simulink library "Cassie_CommandBlock_Library_6"  (R2017b)
settings: Solver=VariableStepAuto  StartTime=0.0  StopTime=10.0  RelTol=1e-3
undefined symbols (not defined in the file): dq, isSim, q, sample_time
libraries: slrtlib x119, Cassie_CommandBlock_Library_5 x1
(part 2 of 3)

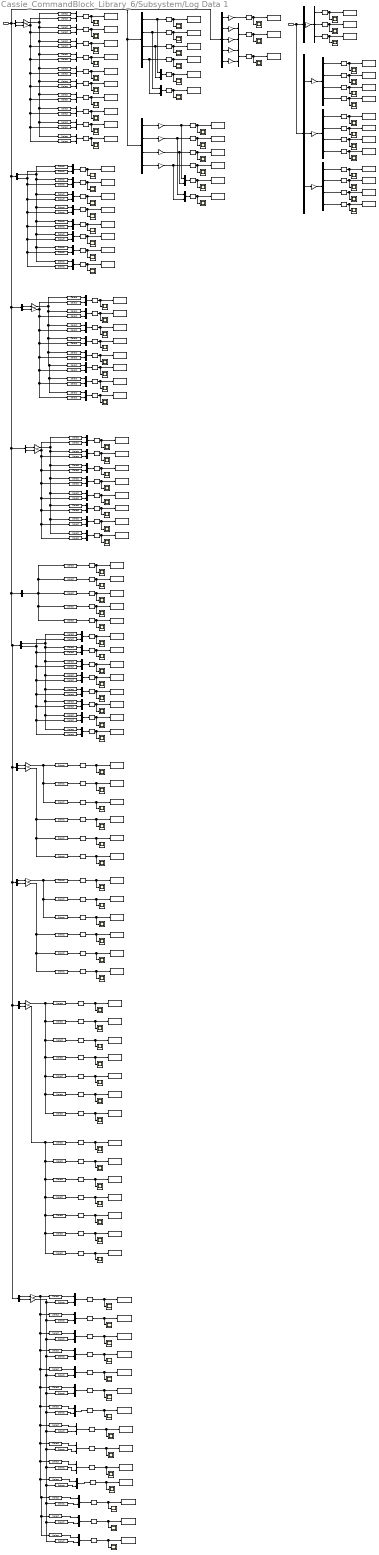
== system Cassie_CommandBlock_Library_6/Subsystem/Log Data 1 ==
  In1 : Inport
  In2 : Inport  Port=2  OutDataTypeStr=Bus: StateEstimator_DataBus
  Bus Selector : BusSelector  OutputSignals=qm0,qmd
  Bus Selector1 : BusSelector  OutputSignals=hr,hr_recover
  Bus Selector10 : BusSelector  OutputSignals=rp_LToe,rp_RToe,rp_LToe_fil,rp_RToe_fil
  Bus Selector11 : BusSelector  OutputSignals=s,qsL_1,qsR_1,qsL_2,qsR_2
  Bus Selector12 : BusSelector  OutputSignals=dq,dq_ss
  Bus Selector13 : BusSelector  OutputSignals=a_world
  Bus Selector14 : BusSelector  OutputSignals=ITx_kf,ITy_kf,ITz_kf
  Bus Selector2 : BusSelector  OutputSignals=hr,h0
  Bus Selector3 : BusSelector  OutputSignals=qd_control,q0_control
  Bus Selector4 : BusSelector  OutputSignals=dqd_control,dq0_control
  Bus Selector5 : BusSelector  OutputSignals=u
  Bus Selector6 : BusSelector  OutputSignals=q,dq
  Bus Selector7 : BusSelector  OutputSignals=q,dq
  Bus Selector8 : BusSelector  OutputSignals=q,dq
  Bus Selector9 : BusSelector  OutputSignals=Lx_stToe_stTD0_obs,Ly_stToe_stTD0_obs,Lx_stToe_stTD0_kf,Ly_stToe_stTD0_kf
  Demux : Demux  Outputs=3
  Demux1 : Demux
  Demux2 : Demux
  Demux3 : Demux
  Gain{,1..4,16..17,24..26} (10 alike) : Gain  Gain=1000
  Gain{5..8,10..15,18..23} (16 alike) : Gain  Gain=180/pi
  Gain9 : Gain  Gain=10
  Mux{,1..61} (62 alike) : Mux  Inputs=2
  Reshape{,1..116} (117 alike) : Reshape
  Scope{,1..116} (117 alike) : Scope
  "Scope " : slrtlib/Displays and Logging/Scope   scopeno=101  scopetype=Host  autostart=on  viewmode=Graphical redraw  formatstr='%15.6f'  grid=on  ylimits=[0,0]  nosamples=250  noprepostsamples=0  interleave=1  triggermode=FreeRun  triggersignal=1  trigsignalfromport=off  triggerlevel=0.0  triggerslope=Either  triggerscope=1  triggersample=0  filename=data.dat  mode=Lazy  writesize=512  autorestart=off  dynamicfilemode=off  maxwritefilesize=512*1024^2
  Scope 1 : slrtlib/Displays and Logging/Scope   scopeno=102  scopetype=Host  autostart=on  viewmode=Graphical redraw  formatstr='%15.6f'  grid=on  ylimits=[0,0]  nosamples=2500  noprepostsamples=0  interleave=1  triggermode=FreeRun  triggersignal=1  trigsignalfromport=off  triggerlevel=0.0  triggerslope=Either  triggerscope=1  triggersample=0  filename=data.dat  mode=Lazy  writesize=512  autorestart=off  dynamicfilemode=off  maxwritefilesize=512*1024^2
  Scope 10 : slrtlib/Displays and Logging/Scope   scopeno=111  scopetype=Host  autostart=on  viewmode=Graphical redraw  formatstr='%15.6f'  grid=on  ylimits=[0,0]  nosamples=2500  noprepostsamples=0  interleave=1  triggermode=FreeRun  triggersignal=1  trigsignalfromport=off  triggerlevel=0.0  triggerslope=Either  triggerscope=1  triggersample=0  filename=data.dat  mode=Lazy  writesize=512  autorestart=off  dynamicfilemode=off  maxwritefilesize=512*1024^2
  Scope 100 : slrtlib/Displays and Logging/Scope   scopeno=501  scopetype=Host  autostart=on  viewmode=Graphical redraw  formatstr='%15.6f'  grid=on  ylimits=[0,0]  nosamples=2500  noprepostsamples=0  interleave=1  triggermode=FreeRun  triggersignal=1  trigsignalfromport=off  triggerlevel=0.0  triggerslope=Either  triggerscope=1  triggersample=0  filename=data.dat  mode=Lazy  writesize=512  autorestart=off  dynamicfilemode=off  maxwritefilesize=512*1024^2
  Scope 101 : slrtlib/Displays and Logging/Scope   scopeno=502  scopetype=Host  autostart=on  viewmode=Graphical redraw  formatstr='%15.6f'  grid=on  ylimits=[0,0]  nosamples=2500  noprepostsamples=0  interleave=1  triggermode=FreeRun  triggersignal=1  trigsignalfromport=off  triggerlevel=0.0  triggerslope=Either  triggerscope=1  triggersample=0  filename=data.dat  mode=Lazy  writesize=512  autorestart=off  dynamicfilemode=off  maxwritefilesize=512*1024^2
  Scope 102 : slrtlib/Displays and Logging/Scope   scopeno=503  scopetype=Host  autostart=on  viewmode=Graphical redraw  formatstr='%15.6f'  grid=on  ylimits=[0,0]  nosamples=2500  noprepostsamples=0  interleave=1  triggermode=FreeRun  triggersignal=1  trigsignalfromport=off  triggerlevel=0.0  triggerslope=Either  triggerscope=1  triggersample=0  filename=data.dat  mode=Lazy  writesize=512  autorestart=off  dynamicfilemode=off  maxwritefilesize=512*1024^2
  Scope 103 : slrtlib/Displays and Logging/Scope   scopeno=403  scopetype=Host  autostart=on  viewmode=Graphical redraw  formatstr='%15.6f'  grid=on  ylimits=[0,0]  nosamples=2500  noprepostsamples=0  interleave=1  triggermode=FreeRun  triggersignal=1  trigsignalfromport=off  triggerlevel=0.0  triggerslope=Either  triggerscope=1  triggersample=0  filename=data.dat  mode=Lazy  writesize=512  autorestart=off  dynamicfilemode=off  maxwritefilesize=512*1024^2
  Scope 104 : slrtlib/Displays and Logging/Scope   scopeno=404  scopetype=Host  autostart=on  viewmode=Graphical redraw  formatstr='%15.6f'  grid=on  ylimits=[0,0]  nosamples=2500  noprepostsamples=0  interleave=1  triggermode=FreeRun  triggersignal=1  trigsignalfromport=off  triggerlevel=0.0  triggerslope=Either  triggerscope=1  triggersample=0  filename=data.dat  mode=Lazy  writesize=512  autorestart=off  dynamicfilemode=off  maxwritefilesize=512*1024^2
  Scope 105 : slrtlib/Displays and Logging/Scope   scopeno=511  scopetype=Host  autostart=on  viewmode=Graphical redraw  formatstr='%15.6f'  grid=on  ylimits=[0,0]  nosamples=2500  noprepostsamples=0  interleave=1  triggermode=FreeRun  triggersignal=1  trigsignalfromport=off  triggerlevel=0.0  triggerslope=Either  triggerscope=1  triggersample=0  filename=data.dat  mode=Lazy  writesize=512  autorestart=off  dynamicfilemode=off  maxwritefilesize=512*1024^2
  Scope 106 : slrtlib/Displays and Logging/Scope   scopeno=512  scopetype=Host  autostart=on  viewmode=Graphical redraw  formatstr='%15.6f'  grid=on  ylimits=[0,0]  nosamples=2500  noprepostsamples=0  interleave=1  triggermode=FreeRun  triggersignal=1  trigsignalfromport=off  triggerlevel=0.0  triggerslope=Either  triggerscope=1  triggersample=0  filename=data.dat  mode=Lazy  writesize=512  autorestart=off  dynamicfilemode=off  maxwritefilesize=512*1024^2
  Scope 107 : slrtlib/Displays and Logging/Scope   scopeno=513  scopetype=Host  autostart=on  viewmode=Graphical redraw  formatstr='%15.6f'  grid=on  ylimits=[0,0]  nosamples=2500  noprepostsamples=0  interleave=1  triggermode=FreeRun  triggersignal=1  trigsignalfromport=off  triggerlevel=0.0  triggerslope=Either  triggerscope=1  triggersample=0  filename=data.dat  mode=Lazy  writesize=512  autorestart=off  dynamicfilemode=off  maxwritefilesize=512*1024^2
  Scope 108 : slrtlib/Displays and Logging/Scope   scopeno=514  scopetype=Host  autostart=on  viewmode=Graphical redraw  formatstr='%15.6f'  grid=on  ylimits=[0,0]  nosamples=2500  noprepostsamples=0  interleave=1  triggermode=FreeRun  triggersignal=1  trigsignalfromport=off  triggerlevel=0.0  triggerslope=Either  triggerscope=1  triggersample=0  filename=data.dat  mode=Lazy  writesize=512  autorestart=off  dynamicfilemode=off  maxwritefilesize=512*1024^2
  Scope 109 : slrtlib/Displays and Logging/Scope   scopeno=515  scopetype=Host  autostart=on  viewmode=Graphical redraw  formatstr='%15.6f'  grid=on  ylimits=[0,0]  nosamples=2500  noprepostsamples=0  interleave=1  triggermode=FreeRun  triggersignal=1  trigsignalfromport=off  triggerlevel=0.0  triggerslope=Either  triggerscope=1  triggersample=0  filename=data.dat  mode=Lazy  writesize=512  autorestart=off  dynamicfilemode=off  maxwritefilesize=512*1024^2
  Scope 11 : slrtlib/Displays and Logging/Scope   scopeno=112  scopetype=Host  autostart=on  viewmode=Graphical redraw  formatstr='%15.6f'  grid=on  ylimits=[0,0]  nosamples=2500  noprepostsamples=0  interleave=1  triggermode=FreeRun  triggersignal=1  trigsignalfromport=off  triggerlevel=0.0  triggerslope=Either  triggerscope=1  triggersample=0  filename=data.dat  mode=Lazy  writesize=512  autorestart=off  dynamicfilemode=off  maxwritefilesize=512*1024^2
  Scope 110 : slrtlib/Displays and Logging/Scope   scopeno=516  scopetype=Host  autostart=on  viewmode=Graphical redraw  formatstr='%15.6f'  grid=on  ylimits=[0,0]  nosamples=2500  noprepostsamples=0  interleave=1  triggermode=FreeRun  triggersignal=1  trigsignalfromport=off  triggerlevel=0.0  triggerslope=Either  triggerscope=1  triggersample=0  filename=data.dat  mode=Lazy  writesize=512  autorestart=off  dynamicfilemode=off  maxwritefilesize=512*1024^2
  Scope 111 : slrtlib/Displays and Logging/Scope   scopeno=517  scopetype=Host  autostart=on  viewmode=Graphical redraw  formatstr='%15.6f'  grid=on  ylimits=[0,0]  nosamples=2500  noprepostsamples=0  interleave=1  triggermode=FreeRun  triggersignal=1  trigsignalfromport=off  triggerlevel=0.0  triggerslope=Either  triggerscope=1  triggersample=0  filename=data.dat  mode=Lazy  writesize=512  autorestart=off  dynamicfilemode=off  maxwritefilesize=512*1024^2
  Scope 112 : slrtlib/Displays and Logging/Scope   scopeno=518  scopetype=Host  autostart=on  viewmode=Graphical redraw  formatstr='%15.6f'  grid=on  ylimits=[0,0]  nosamples=2500  noprepostsamples=0  interleave=1  triggermode=FreeRun  triggersignal=1  trigsignalfromport=off  triggerlevel=0.0  triggerslope=Either  triggerscope=1  triggersample=0  filename=data.dat  mode=Lazy  writesize=512  autorestart=off  dynamicfilemode=off  maxwritefilesize=512*1024^2
  Scope 113 : slrtlib/Displays and Logging/Scope   scopeno=519  scopetype=Host  autostart=on  viewmode=Graphical redraw  formatstr='%15.6f'  grid=on  ylimits=[0,0]  nosamples=2500  noprepostsamples=0  interleave=1  triggermode=FreeRun  triggersignal=1  trigsignalfromport=off  triggerlevel=0.0  triggerslope=Either  triggerscope=1  triggersample=0  filename=data.dat  mode=Lazy  writesize=512  autorestart=off  dynamicfilemode=off  maxwritefilesize=512*1024^2
  Scope 114 : slrtlib/Displays and Logging/Scope   scopeno=520  scopetype=Host  autostart=on  viewmode=Graphical redraw  formatstr='%15.6f'  grid=on  ylimits=[0,0]  nosamples=2500  noprepostsamples=0  interleave=1  triggermode=FreeRun  triggersignal=1  trigsignalfromport=off  triggerlevel=0.0  triggerslope=Either  triggerscope=1  triggersample=0  filename=data.dat  mode=Lazy  writesize=512  autorestart=off  dynamicfilemode=off  maxwritefilesize=512*1024^2
  Scope 115 : slrtlib/Displays and Logging/Scope   scopeno=521  scopetype=Host  autostart=on  viewmode=Graphical redraw  formatstr='%15.6f'  grid=on  ylimits=[0,0]  nosamples=2500  noprepostsamples=0  interleave=1  triggermode=FreeRun  triggersignal=1  trigsignalfromport=off  triggerlevel=0.0  triggerslope=Either  triggerscope=1  triggersample=0  filename=data.dat  mode=Lazy  writesize=512  autorestart=off  dynamicfilemode=off  maxwritefilesize=512*1024^2
  Scope 116 : slrtlib/Displays and Logging/Scope   scopeno=522  scopetype=Host  autostart=on  viewmode=Graphical redraw  formatstr='%15.6f'  grid=on  ylimits=[0,0]  nosamples=2500  noprepostsamples=0  interleave=1  triggermode=FreeRun  triggersignal=1  trigsignalfromport=off  triggerlevel=0.0  triggerslope=Either  triggerscope=1  triggersample=0  filename=data.dat  mode=Lazy  writesize=512  autorestart=off  dynamicfilemode=off  maxwritefilesize=512*1024^2
  Scope 12 : slrtlib/Displays and Logging/Scope   scopeno=113  scopetype=Host  autostart=on  viewmode=Graphical redraw  formatstr='%15.6f'  grid=on  ylimits=[0,0]  nosamples=2500  noprepostsamples=0  interleave=1  triggermode=FreeRun  triggersignal=1  trigsignalfromport=off  triggerlevel=0.0  triggerslope=Either  triggerscope=1  triggersample=0  filename=data.dat  mode=Lazy  writesize=512  autorestart=off  dynamicfilemode=off  maxwritefilesize=512*1024^2
  Scope 13 : slrtlib/Displays and Logging/Scope   scopeno=114  scopetype=Host  autostart=on  viewmode=Graphical redraw  formatstr='%15.6f'  grid=on  ylimits=[0,0]  nosamples=2500  noprepostsamples=0  interleave=1  triggermode=FreeRun  triggersignal=1  trigsignalfromport=off  triggerlevel=0.0  triggerslope=Either  triggerscope=1  triggersample=0  filename=data.dat  mode=Lazy  writesize=512  autorestart=off  dynamicfilemode=off  maxwritefilesize=512*1024^2
  Scope 14 : slrtlib/Displays and Logging/Scope   scopeno=115  scopetype=Host  autostart=on  viewmode=Graphical redraw  formatstr='%15.6f'  grid=on  ylimits=[0,0]  nosamples=2500  noprepostsamples=0  interleave=1  triggermode=FreeRun  triggersignal=1  trigsignalfromport=off  triggerlevel=0.0  triggerslope=Either  triggerscope=1  triggersample=0  filename=data.dat  mode=Lazy  writesize=512  autorestart=off  dynamicfilemode=off  maxwritefilesize=512*1024^2
  Scope 15 : slrtlib/Displays and Logging/Scope   scopeno=116  scopetype=Host  autostart=on  viewmode=Graphical redraw  formatstr='%15.6f'  grid=on  ylimits=[0,0]  nosamples=2500  noprepostsamples=0  interleave=1  triggermode=FreeRun  triggersignal=1  trigsignalfromport=off  triggerlevel=0.0  triggerslope=Either  triggerscope=1  triggersample=0  filename=data.dat  mode=Lazy  writesize=512  autorestart=off  dynamicfilemode=off  maxwritefilesize=512*1024^2
  Scope 16 : slrtlib/Displays and Logging/Scope   scopeno=117  scopetype=Host  autostart=on  viewmode=Graphical redraw  formatstr='%15.6f'  grid=on  ylimits=[0,0]  nosamples=2500  noprepostsamples=0  interleave=1  triggermode=FreeRun  triggersignal=1  trigsignalfromport=off  triggerlevel=0.0  triggerslope=Either  triggerscope=1  triggersample=0  filename=data.dat  mode=Lazy  writesize=512  autorestart=off  dynamicfilemode=off  maxwritefilesize=512*1024^2
  Scope 17 : slrtlib/Displays and Logging/Scope   scopeno=118  scopetype=Host  autostart=on  viewmode=Graphical redraw  formatstr='%15.6f'  grid=on  ylimits=[0,0]  nosamples=2500  noprepostsamples=0  interleave=1  triggermode=FreeRun  triggersignal=1  trigsignalfromport=off  triggerlevel=0.0  triggerslope=Either  triggerscope=1  triggersample=0  filename=data.dat  mode=Lazy  writesize=512  autorestart=off  dynamicfilemode=off  maxwritefilesize=512*1024^2
  Scope 18 : slrtlib/Displays and Logging/Scope   scopeno=131  scopetype=Host  autostart=on  viewmode=Graphical redraw  formatstr='%15.6f'  grid=on  ylimits=[0,0]  nosamples=2500  noprepostsamples=0  interleave=1  triggermode=FreeRun  triggersignal=1  trigsignalfromport=off  triggerlevel=0.0  triggerslope=Either  triggerscope=1  triggersample=0  filename=data.dat  mode=Lazy  writesize=512  autorestart=off  dynamicfilemode=off  maxwritefilesize=512*1024^2
  Scope 19 : slrtlib/Displays and Logging/Scope   scopeno=132  scopetype=Host  autostart=on  viewmode=Graphical redraw  formatstr='%15.6f'  grid=on  ylimits=[0,0]  nosamples=2500  noprepostsamples=0  interleave=1  triggermode=FreeRun  triggersignal=1  trigsignalfromport=off  triggerlevel=0.0  triggerslope=Either  triggerscope=1  triggersample=0  filename=data.dat  mode=Lazy  writesize=512  autorestart=off  dynamicfilemode=off  maxwritefilesize=512*1024^2
  Scope 2 : slrtlib/Displays and Logging/Scope   scopeno=103  scopetype=Host  autostart=on  viewmode=Graphical redraw  formatstr='%15.6f'  grid=on  ylimits=[0,0]  nosamples=2500  noprepostsamples=0  interleave=1  triggermode=FreeRun  triggersignal=1  trigsignalfromport=off  triggerlevel=0.0  triggerslope=Either  triggerscope=1  triggersample=0  filename=data.dat  mode=Lazy  writesize=512  autorestart=off  dynamicfilemode=off  maxwritefilesize=512*1024^2
  Scope 20 : slrtlib/Displays and Logging/Scope   scopeno=133  scopetype=Host  autostart=on  viewmode=Graphical redraw  formatstr='%15.6f'  grid=on  ylimits=[0,0]  nosamples=2500  noprepostsamples=0  interleave=1  triggermode=FreeRun  triggersignal=1  trigsignalfromport=off  triggerlevel=0.0  triggerslope=Either  triggerscope=1  triggersample=0  filename=data.dat  mode=Lazy  writesize=512  autorestart=off  dynamicfilemode=off  maxwritefilesize=512*1024^2
  Scope 21 : slrtlib/Displays and Logging/Scope   scopeno=134  scopetype=Host  autostart=on  viewmode=Graphical redraw  formatstr='%15.6f'  grid=on  ylimits=[0,0]  nosamples=2500  noprepostsamples=0  interleave=1  triggermode=FreeRun  triggersignal=1  trigsignalfromport=off  triggerlevel=0.0  triggerslope=Either  triggerscope=1  triggersample=0  filename=data.dat  mode=Lazy  writesize=512  autorestart=off  dynamicfilemode=off  maxwritefilesize=512*1024^2
  Scope 22 : slrtlib/Displays and Logging/Scope   scopeno=135  scopetype=Host  autostart=on  viewmode=Graphical redraw  formatstr='%15.6f'  grid=on  ylimits=[0,0]  nosamples=2500  noprepostsamples=0  interleave=1  triggermode=FreeRun  triggersignal=1  trigsignalfromport=off  triggerlevel=0.0  triggerslope=Either  triggerscope=1  triggersample=0  filename=data.dat  mode=Lazy  writesize=512  autorestart=off  dynamicfilemode=off  maxwritefilesize=512*1024^2
  Scope 23 : slrtlib/Displays and Logging/Scope   scopeno=136  scopetype=Host  autostart=on  viewmode=Graphical redraw  formatstr='%15.6f'  grid=on  ylimits=[0,0]  nosamples=2500  noprepostsamples=0  interleave=1  triggermode=FreeRun  triggersignal=1  trigsignalfromport=off  triggerlevel=0.0  triggerslope=Either  triggerscope=1  triggersample=0  filename=data.dat  mode=Lazy  writesize=512  autorestart=off  dynamicfilemode=off  maxwritefilesize=512*1024^2
  Scope 24 : slrtlib/Displays and Logging/Scope   scopeno=137  scopetype=Host  autostart=on  viewmode=Graphical redraw  formatstr='%15.6f'  grid=on  ylimits=[0,0]  nosamples=2500  noprepostsamples=0  interleave=1  triggermode=FreeRun  triggersignal=1  trigsignalfromport=off  triggerlevel=0.0  triggerslope=Either  triggerscope=1  triggersample=0  filename=data.dat  mode=Lazy  writesize=512  autorestart=off  dynamicfilemode=off  maxwritefilesize=512*1024^2
  Scope 25 : slrtlib/Displays and Logging/Scope   scopeno=138  scopetype=Host  autostart=on  viewmode=Graphical redraw  formatstr='%15.6f'  grid=on  ylimits=[0,0]  nosamples=2500  noprepostsamples=0  interleave=1  triggermode=FreeRun  triggersignal=1  trigsignalfromport=off  triggerlevel=0.0  triggerslope=Either  triggerscope=1  triggersample=0  filename=data.dat  mode=Lazy  writesize=512  autorestart=off  dynamicfilemode=off  maxwritefilesize=512*1024^2
  Scope 26 : slrtlib/Displays and Logging/Scope   scopeno=141  scopetype=Host  autostart=on  viewmode=Graphical redraw  formatstr='%15.6f'  grid=on  ylimits=[0,0]  nosamples=2500  noprepostsamples=0  interleave=1  triggermode=FreeRun  triggersignal=1  trigsignalfromport=off  triggerlevel=0.0  triggerslope=Either  triggerscope=1  triggersample=0  filename=data.dat  mode=Lazy  writesize=512  autorestart=off  dynamicfilemode=off  maxwritefilesize=512*1024^2
  Scope 27 : slrtlib/Displays and Logging/Scope   scopeno=142  scopetype=Host  autostart=on  viewmode=Graphical redraw  formatstr='%15.6f'  grid=on  ylimits=[0,0]  nosamples=2500  noprepostsamples=0  interleave=1  triggermode=FreeRun  triggersignal=1  trigsignalfromport=off  triggerlevel=0.0  triggerslope=Either  triggerscope=1  triggersample=0  filename=data.dat  mode=Lazy  writesize=512  autorestart=off  dynamicfilemode=off  maxwritefilesize=512*1024^2
  Scope 28 : slrtlib/Displays and Logging/Scope   scopeno=143  scopetype=Host  autostart=on  viewmode=Graphical redraw  formatstr='%15.6f'  grid=on  ylimits=[0,0]  nosamples=2500  noprepostsamples=0  interleave=1  triggermode=FreeRun  triggersignal=1  trigsignalfromport=off  triggerlevel=0.0  triggerslope=Either  triggerscope=1  triggersample=0  filename=data.dat  mode=Lazy  writesize=512  autorestart=off  dynamicfilemode=off  maxwritefilesize=512*1024^2
  Scope 29 : slrtlib/Displays and Logging/Scope   scopeno=144  scopetype=Host  autostart=on  viewmode=Graphical redraw  formatstr='%15.6f'  grid=on  ylimits=[0,0]  nosamples=2500  noprepostsamples=0  interleave=1  triggermode=FreeRun  triggersignal=1  trigsignalfromport=off  triggerlevel=0.0  triggerslope=Either  triggerscope=1  triggersample=0  filename=data.dat  mode=Lazy  writesize=512  autorestart=off  dynamicfilemode=off  maxwritefilesize=512*1024^2
  Scope 3 : slrtlib/Displays and Logging/Scope   scopeno=104  scopetype=Host  autostart=on  viewmode=Graphical redraw  formatstr='%15.6f'  grid=on  ylimits=[0,0]  nosamples=2500  noprepostsamples=0  interleave=1  triggermode=FreeRun  triggersignal=1  trigsignalfromport=off  triggerlevel=0.0  triggerslope=Either  triggerscope=1  triggersample=0  filename=data.dat  mode=Lazy  writesize=512  autorestart=off  dynamicfilemode=off  maxwritefilesize=512*1024^2
  Scope 30 : slrtlib/Displays and Logging/Scope   scopeno=145  scopetype=Host  autostart=on  viewmode=Graphical redraw  formatstr='%15.6f'  grid=on  ylimits=[0,0]  nosamples=2500  noprepostsamples=0  interleave=1  triggermode=FreeRun  triggersignal=1  trigsignalfromport=off  triggerlevel=0.0  triggerslope=Either  triggerscope=1  triggersample=0  filename=data.dat  mode=Lazy  writesize=512  autorestart=off  dynamicfilemode=off  maxwritefilesize=512*1024^2
  Scope 31 : slrtlib/Displays and Logging/Scope   scopeno=146  scopetype=Host  autostart=on  viewmode=Graphical redraw  formatstr='%15.6f'  grid=on  ylimits=[0,0]  nosamples=2500  noprepostsamples=0  interleave=1  triggermode=FreeRun  triggersignal=1  trigsignalfromport=off  triggerlevel=0.0  triggerslope=Either  triggerscope=1  triggersample=0  filename=data.dat  mode=Lazy  writesize=512  autorestart=off  dynamicfilemode=off  maxwritefilesize=512*1024^2
  Scope 32 : slrtlib/Displays and Logging/Scope   scopeno=147  scopetype=Host  autostart=on  viewmode=Graphical redraw  formatstr='%15.6f'  grid=on  ylimits=[0,0]  nosamples=2500  noprepostsamples=0  interleave=1  triggermode=FreeRun  triggersignal=1  trigsignalfromport=off  triggerlevel=0.0  triggerslope=Either  triggerscope=1  triggersample=0  filename=data.dat  mode=Lazy  writesize=512  autorestart=off  dynamicfilemode=off  maxwritefilesize=512*1024^2
  Scope 33 : slrtlib/Displays and Logging/Scope   scopeno=148  scopetype=Host  autostart=on  viewmode=Graphical redraw  formatstr='%15.6f'  grid=on  ylimits=[0,0]  nosamples=2500  noprepostsamples=0  interleave=1  triggermode=FreeRun  triggersignal=1  trigsignalfromport=off  triggerlevel=0.0  triggerslope=Either  triggerscope=1  triggersample=0  filename=data.dat  mode=Lazy  writesize=512  autorestart=off  dynamicfilemode=off  maxwritefilesize=512*1024^2
  Scope 34 : slrtlib/Displays and Logging/Scope   scopeno=161  scopetype=Host  autostart=on  viewmode=Graphical redraw  formatstr='%15.6f'  grid=on  ylimits=[0,0]  nosamples=2500  noprepostsamples=0  interleave=1  triggermode=FreeRun  triggersignal=1  trigsignalfromport=off  triggerlevel=0.0  triggerslope=Either  triggerscope=1  triggersample=0  filename=data.dat  mode=Lazy  writesize=512  autorestart=off  dynamicfilemode=off  maxwritefilesize=512*1024^2
  Scope 35 : slrtlib/Displays and Logging/Scope   scopeno=162  scopetype=Host  autostart=on  viewmode=Graphical redraw  formatstr='%15.6f'  grid=on  ylimits=[0,0]  nosamples=2500  noprepostsamples=0  interleave=1  triggermode=FreeRun  triggersignal=1  trigsignalfromport=off  triggerlevel=0.0  triggerslope=Either  triggerscope=1  triggersample=0  filename=data.dat  mode=Lazy  writesize=512  autorestart=off  dynamicfilemode=off  maxwritefilesize=512*1024^2
  Scope 36 : slrtlib/Displays and Logging/Scope   scopeno=163  scopetype=Host  autostart=on  viewmode=Graphical redraw  formatstr='%15.6f'  grid=on  ylimits=[0,0]  nosamples=2500  noprepostsamples=0  interleave=1  triggermode=FreeRun  triggersignal=1  trigsignalfromport=off  triggerlevel=0.0  triggerslope=Either  triggerscope=1  triggersample=0  filename=data.dat  mode=Lazy  writesize=512  autorestart=off  dynamicfilemode=off  maxwritefilesize=512*1024^2
  Scope 37 : slrtlib/Displays and Logging/Scope   scopeno=164  scopetype=Host  autostart=on  viewmode=Graphical redraw  formatstr='%15.6f'  grid=on  ylimits=[0,0]  nosamples=2500  noprepostsamples=0  interleave=1  triggermode=FreeRun  triggersignal=1  trigsignalfromport=off  triggerlevel=0.0  triggerslope=Either  triggerscope=1  triggersample=0  filename=data.dat  mode=Lazy  writesize=512  autorestart=off  dynamicfilemode=off  maxwritefilesize=512*1024^2
  Scope 38 : slrtlib/Displays and Logging/Scope   scopeno=165  scopetype=Host  autostart=on  viewmode=Graphical redraw  formatstr='%15.6f'  grid=on  ylimits=[0,0]  nosamples=2500  noprepostsamples=0  interleave=1  triggermode=FreeRun  triggersignal=1  trigsignalfromport=off  triggerlevel=0.0  triggerslope=Either  triggerscope=1  triggersample=0  filename=data.dat  mode=Lazy  writesize=512  autorestart=off  dynamicfilemode=off  maxwritefilesize=512*1024^2
  Scope 39 : slrtlib/Displays and Logging/Scope   scopeno=166  scopetype=Host  autostart=on  viewmode=Graphical redraw  formatstr='%15.6f'  grid=on  ylimits=[0,0]  nosamples=2500  noprepostsamples=0  interleave=1  triggermode=FreeRun  triggersignal=1  trigsignalfromport=off  triggerlevel=0.0  triggerslope=Either  triggerscope=1  triggersample=0  filename=data.dat  mode=Lazy  writesize=512  autorestart=off  dynamicfilemode=off  maxwritefilesize=512*1024^2
  Scope 4 : slrtlib/Displays and Logging/Scope   scopeno=105  scopetype=Host  autostart=on  viewmode=Graphical redraw  formatstr='%15.6f'  grid=on  ylimits=[0,0]  nosamples=2500  noprepostsamples=0  interleave=1  triggermode=FreeRun  triggersignal=1  trigsignalfromport=off  triggerlevel=0.0  triggerslope=Either  triggerscope=1  triggersample=0  filename=data.dat  mode=Lazy  writesize=512  autorestart=off  dynamicfilemode=off  maxwritefilesize=512*1024^2
  Scope 40 : slrtlib/Displays and Logging/Scope   scopeno=151  scopetype=Host  autostart=on  viewmode=Graphical redraw  formatstr='%15.6f'  grid=on  ylimits=[0,0]  nosamples=2500  noprepostsamples=0  interleave=1  triggermode=FreeRun  triggersignal=1  trigsignalfromport=off  triggerlevel=0.0  triggerslope=Either  triggerscope=1  triggersample=0  filename=data.dat  mode=Lazy  writesize=512  autorestart=off  dynamicfilemode=off  maxwritefilesize=512*1024^2
  Scope 41 : slrtlib/Displays and Logging/Scope   scopeno=152  scopetype=Host  autostart=on  viewmode=Graphical redraw  formatstr='%15.6f'  grid=on  ylimits=[0,0]  nosamples=2500  noprepostsamples=0  interleave=1  triggermode=FreeRun  triggersignal=1  trigsignalfromport=off  triggerlevel=0.0  triggerslope=Either  triggerscope=1  triggersample=0  filename=data.dat  mode=Lazy  writesize=512  autorestart=off  dynamicfilemode=off  maxwritefilesize=512*1024^2
  Scope 42 : slrtlib/Displays and Logging/Scope   scopeno=153  scopetype=Host  autostart=on  viewmode=Graphical redraw  formatstr='%15.6f'  grid=on  ylimits=[0,0]  nosamples=2500  noprepostsamples=0  interleave=1  triggermode=FreeRun  triggersignal=1  trigsignalfromport=off  triggerlevel=0.0  triggerslope=Either  triggerscope=1  triggersample=0  filename=data.dat  mode=Lazy  writesize=512  autorestart=off  dynamicfilemode=off  maxwritefilesize=512*1024^2
  Scope 43 : slrtlib/Displays and Logging/Scope   scopeno=154  scopetype=Host  autostart=on  viewmode=Graphical redraw  formatstr='%15.6f'  grid=on  ylimits=[0,0]  nosamples=2500  noprepostsamples=0  interleave=1  triggermode=FreeRun  triggersignal=1  trigsignalfromport=off  triggerlevel=0.0  triggerslope=Either  triggerscope=1  triggersample=0  filename=data.dat  mode=Lazy  writesize=512  autorestart=off  dynamicfilemode=off  maxwritefilesize=512*1024^2
  Scope 44 : slrtlib/Displays and Logging/Scope   scopeno=155  scopetype=Host  autostart=on  viewmode=Graphical redraw  formatstr='%15.6f'  grid=on  ylimits=[0,0]  nosamples=2500  noprepostsamples=0  interleave=1  triggermode=FreeRun  triggersignal=1  trigsignalfromport=off  triggerlevel=0.0  triggerslope=Either  triggerscope=1  triggersample=0  filename=data.dat  mode=Lazy  writesize=512  autorestart=off  dynamicfilemode=off  maxwritefilesize=512*1024^2
  Scope 45 : slrtlib/Displays and Logging/Scope   scopeno=167  scopetype=Host  autostart=on  viewmode=Graphical redraw  formatstr='%15.6f'  grid=on  ylimits=[0,0]  nosamples=2500  noprepostsamples=0  interleave=1  triggermode=FreeRun  triggersignal=1  trigsignalfromport=off  triggerlevel=0.0  triggerslope=Either  triggerscope=1  triggersample=0  filename=data.dat  mode=Lazy  writesize=512  autorestart=off  dynamicfilemode=off  maxwritefilesize=512*1024^2
  Scope 46 : slrtlib/Displays and Logging/Scope   scopeno=168  scopetype=Host  autostart=on  viewmode=Graphical redraw  formatstr='%15.6f'  grid=on  ylimits=[0,0]  nosamples=2500  noprepostsamples=0  interleave=1  triggermode=FreeRun  triggersignal=1  trigsignalfromport=off  triggerlevel=0.0  triggerslope=Either  triggerscope=1  triggersample=0  filename=data.dat  mode=Lazy  writesize=512  autorestart=off  dynamicfilemode=off  maxwritefilesize=512*1024^2
  Scope 47 : slrtlib/Displays and Logging/Scope   scopeno=171  scopetype=Host  autostart=on  viewmode=Graphical redraw  formatstr='%15.6f'  grid=on  ylimits=[0,0]  nosamples=2500  noprepostsamples=0  interleave=1  triggermode=FreeRun  triggersignal=1  trigsignalfromport=off  triggerlevel=0.0  triggerslope=Either  triggerscope=1  triggersample=0  filename=data.dat  mode=Lazy  writesize=512  autorestart=off  dynamicfilemode=off  maxwritefilesize=512*1024^2
  Scope 48 : slrtlib/Displays and Logging/Scope   scopeno=172  scopetype=Host  autostart=on  viewmode=Graphical redraw  formatstr='%15.6f'  grid=on  ylimits=[0,0]  nosamples=2500  noprepostsamples=0  interleave=1  triggermode=FreeRun  triggersignal=1  trigsignalfromport=off  triggerlevel=0.0  triggerslope=Either  triggerscope=1  triggersample=0  filename=data.dat  mode=Lazy  writesize=512  autorestart=off  dynamicfilemode=off  maxwritefilesize=512*1024^2
  Scope 49 : slrtlib/Displays and Logging/Scope   scopeno=173  scopetype=Host  autostart=on  viewmode=Graphical redraw  formatstr='%15.6f'  grid=on  ylimits=[0,0]  nosamples=2500  noprepostsamples=0  interleave=1  triggermode=FreeRun  triggersignal=1  trigsignalfromport=off  triggerlevel=0.0  triggerslope=Either  triggerscope=1  triggersample=0  filename=data.dat  mode=Lazy  writesize=512  autorestart=off  dynamicfilemode=off  maxwritefilesize=512*1024^2
  Scope 5 : slrtlib/Displays and Logging/Scope   scopeno=106  scopetype=Host  autostart=on  viewmode=Graphical redraw  formatstr='%15.6f'  grid=on  ylimits=[0,0]  nosamples=2500  noprepostsamples=0  interleave=1  triggermode=FreeRun  triggersignal=1  trigsignalfromport=off  triggerlevel=0.0  triggerslope=Either  triggerscope=1  triggersample=0  filename=data.dat  mode=Lazy  writesize=512  autorestart=off  dynamicfilemode=off  maxwritefilesize=512*1024^2
  Scope 50 : slrtlib/Displays and Logging/Scope   scopeno=174  scopetype=Host  autostart=on  viewmode=Graphical redraw  formatstr='%15.6f'  grid=on  ylimits=[0,0]  nosamples=2500  noprepostsamples=0  interleave=1  triggermode=FreeRun  triggersignal=1  trigsignalfromport=off  triggerlevel=0.0  triggerslope=Either  triggerscope=1  triggersample=0  filename=data.dat  mode=Lazy  writesize=512  autorestart=off  dynamicfilemode=off  maxwritefilesize=512*1024^2
  Scope 51 : slrtlib/Displays and Logging/Scope   scopeno=175  scopetype=Host  autostart=on  viewmode=Graphical redraw  formatstr='%15.6f'  grid=on  ylimits=[0,0]  nosamples=2500  noprepostsamples=0  interleave=1  triggermode=FreeRun  triggersignal=1  trigsignalfromport=off  triggerlevel=0.0  triggerslope=Either  triggerscope=1  triggersample=0  filename=data.dat  mode=Lazy  writesize=512  autorestart=off  dynamicfilemode=off  maxwritefilesize=512*1024^2
  Scope 52 : slrtlib/Displays and Logging/Scope   scopeno=176  scopetype=Host  autostart=on  viewmode=Graphical redraw  formatstr='%15.6f'  grid=on  ylimits=[0,0]  nosamples=2500  noprepostsamples=0  interleave=1  triggermode=FreeRun  triggersignal=1  trigsignalfromport=off  triggerlevel=0.0  triggerslope=Either  triggerscope=1  triggersample=0  filename=data.dat  mode=Lazy  writesize=512  autorestart=off  dynamicfilemode=off  maxwritefilesize=512*1024^2
  Scope 53 : slrtlib/Displays and Logging/Scope   scopeno=181  scopetype=Host  autostart=on  viewmode=Graphical redraw  formatstr='%15.6f'  grid=on  ylimits=[0,0]  nosamples=2500  noprepostsamples=0  interleave=1  triggermode=FreeRun  triggersignal=1  trigsignalfromport=off  triggerlevel=0.0  triggerslope=Either  triggerscope=1  triggersample=0  filename=data.dat  mode=Lazy  writesize=512  autorestart=off  dynamicfilemode=off  maxwritefilesize=512*1024^2
  Scope 54 : slrtlib/Displays and Logging/Scope   scopeno=182  scopetype=Host  autostart=on  viewmode=Graphical redraw  formatstr='%15.6f'  grid=on  ylimits=[0,0]  nosamples=2500  noprepostsamples=0  interleave=1  triggermode=FreeRun  triggersignal=1  trigsignalfromport=off  triggerlevel=0.0  triggerslope=Either  triggerscope=1  triggersample=0  filename=data.dat  mode=Lazy  writesize=512  autorestart=off  dynamicfilemode=off  maxwritefilesize=512*1024^2
  Scope 55 : slrtlib/Displays and Logging/Scope   scopeno=183  scopetype=Host  autostart=on  viewmode=Graphical redraw  formatstr='%15.6f'  grid=on  ylimits=[0,0]  nosamples=2500  noprepostsamples=0  interleave=1  triggermode=FreeRun  triggersignal=1  trigsignalfromport=off  triggerlevel=0.0  triggerslope=Either  triggerscope=1  triggersample=0  filename=data.dat  mode=Lazy  writesize=512  autorestart=off  dynamicfilemode=off  maxwritefilesize=512*1024^2
  Scope 56 : slrtlib/Displays and Logging/Scope   scopeno=184  scopetype=Host  autostart=on  viewmode=Graphical redraw  formatstr='%15.6f'  grid=on  ylimits=[0,0]  nosamples=2500  noprepostsamples=0  interleave=1  triggermode=FreeRun  triggersignal=1  trigsignalfromport=off  triggerlevel=0.0  triggerslope=Either  triggerscope=1  triggersample=0  filename=data.dat  mode=Lazy  writesize=512  autorestart=off  dynamicfilemode=off  maxwritefilesize=512*1024^2
  Scope 57 : slrtlib/Displays and Logging/Scope   scopeno=185  scopetype=Host  autostart=on  viewmode=Graphical redraw  formatstr='%15.6f'  grid=on  ylimits=[0,0]  nosamples=2500  noprepostsamples=0  interleave=1  triggermode=FreeRun  triggersignal=1  trigsignalfromport=off  triggerlevel=0.0  triggerslope=Either  triggerscope=1  triggersample=0  filename=data.dat  mode=Lazy  writesize=512  autorestart=off  dynamicfilemode=off  maxwritefilesize=512*1024^2
  Scope 58 : slrtlib/Displays and Logging/Scope   scopeno=186  scopetype=Host  autostart=on  viewmode=Graphical redraw  formatstr='%15.6f'  grid=on  ylimits=[0,0]  nosamples=2500  noprepostsamples=0  interleave=1  triggermode=FreeRun  triggersignal=1  trigsignalfromport=off  triggerlevel=0.0  triggerslope=Either  triggerscope=1  triggersample=0  filename=data.dat  mode=Lazy  writesize=512  autorestart=off  dynamicfilemode=off  maxwritefilesize=512*1024^2
  Scope 59 : slrtlib/Displays and Logging/Scope   scopeno=191  scopetype=Host  autostart=on  viewmode=Graphical redraw  formatstr='%15.6f'  grid=on  ylimits=[0,0]  nosamples=2500  noprepostsamples=0  interleave=1  triggermode=FreeRun  triggersignal=1  trigsignalfromport=off  triggerlevel=0.0  triggerslope=Either  triggerscope=1  triggersample=0  filename=data.dat  mode=Lazy  writesize=512  autorestart=off  dynamicfilemode=off  maxwritefilesize=512*1024^2
  Scope 6 : slrtlib/Displays and Logging/Scope   scopeno=107  scopetype=Host  autostart=on  viewmode=Graphical redraw  formatstr='%15.6f'  grid=on  ylimits=[0,0]  nosamples=2500  noprepostsamples=0  interleave=1  triggermode=FreeRun  triggersignal=1  trigsignalfromport=off  triggerlevel=0.0  triggerslope=Either  triggerscope=1  triggersample=0  filename=data.dat  mode=Lazy  writesize=512  autorestart=off  dynamicfilemode=off  maxwritefilesize=512*1024^2
  Scope 60 : slrtlib/Displays and Logging/Scope   scopeno=192  scopetype=Host  autostart=on  viewmode=Graphical redraw  formatstr='%15.6f'  grid=on  ylimits=[0,0]  nosamples=2500  noprepostsamples=0  interleave=1  triggermode=FreeRun  triggersignal=1  trigsignalfromport=off  triggerlevel=0.0  triggerslope=Either  triggerscope=1  triggersample=0  filename=data.dat  mode=Lazy  writesize=512  autorestart=off  dynamicfilemode=off  maxwritefilesize=512*1024^2
  Scope 61 : slrtlib/Displays and Logging/Scope   scopeno=193  scopetype=Host  autostart=on  viewmode=Graphical redraw  formatstr='%15.6f'  grid=on  ylimits=[0,0]  nosamples=2500  noprepostsamples=0  interleave=1  triggermode=FreeRun  triggersignal=1  trigsignalfromport=off  triggerlevel=0.0  triggerslope=Either  triggerscope=1  triggersample=0  filename=data.dat  mode=Lazy  writesize=512  autorestart=off  dynamicfilemode=off  maxwritefilesize=512*1024^2
  Scope 62 : slrtlib/Displays and Logging/Scope   scopeno=194  scopetype=Host  autostart=on  viewmode=Graphical redraw  formatstr='%15.6f'  grid=on  ylimits=[0,0]  nosamples=2500  noprepostsamples=0  interleave=1  triggermode=FreeRun  triggersignal=1  trigsignalfromport=off  triggerlevel=0.0  triggerslope=Either  triggerscope=1  triggersample=0  filename=data.dat  mode=Lazy  writesize=512  autorestart=off  dynamicfilemode=off  maxwritefilesize=512*1024^2
  Scope 63 : slrtlib/Displays and Logging/Scope   scopeno=195  scopetype=Host  autostart=on  viewmode=Graphical redraw  formatstr='%15.6f'  grid=on  ylimits=[0,0]  nosamples=2500  noprepostsamples=0  interleave=1  triggermode=FreeRun  triggersignal=1  trigsignalfromport=off  triggerlevel=0.0  triggerslope=Either  triggerscope=1  triggersample=0  filename=data.dat  mode=Lazy  writesize=512  autorestart=off  dynamicfilemode=off  maxwritefilesize=512*1024^2
  Scope 64 : slrtlib/Displays and Logging/Scope   scopeno=196  scopetype=Host  autostart=on  viewmode=Graphical redraw  formatstr='%15.6f'  grid=on  ylimits=[0,0]  nosamples=2500  noprepostsamples=0  interleave=1  triggermode=FreeRun  triggersignal=1  trigsignalfromport=off  triggerlevel=0.0  triggerslope=Either  triggerscope=1  triggersample=0  filename=data.dat  mode=Lazy  writesize=512  autorestart=off  dynamicfilemode=off  maxwritefilesize=512*1024^2
  Scope 65 : slrtlib/Displays and Logging/Scope   scopeno=197  scopetype=Host  autostart=on  viewmode=Graphical redraw  formatstr='%15.6f'  grid=on  ylimits=[0,0]  nosamples=2500  noprepostsamples=0  interleave=1  triggermode=FreeRun  triggersignal=1  trigsignalfromport=off  triggerlevel=0.0  triggerslope=Either  triggerscope=1  triggersample=0  filename=data.dat  mode=Lazy  writesize=512  autorestart=off  dynamicfilemode=off  maxwritefilesize=512*1024^2
  Scope 66 : slrtlib/Displays and Logging/Scope   scopeno=201  scopetype=Host  autostart=on  viewmode=Graphical redraw  formatstr='%15.6f'  grid=on  ylimits=[0,0]  nosamples=2500  noprepostsamples=0  interleave=1  triggermode=FreeRun  triggersignal=1  trigsignalfromport=off  triggerlevel=0.0  triggerslope=Either  triggerscope=1  triggersample=0  filename=data.dat  mode=Lazy  writesize=512  autorestart=off  dynamicfilemode=off  maxwritefilesize=512*1024^2
  Scope 67 : slrtlib/Displays and Logging/Scope   scopeno=202  scopetype=Host  autostart=on  viewmode=Graphical redraw  formatstr='%15.6f'  grid=on  ylimits=[0,0]  nosamples=2500  noprepostsamples=0  interleave=1  triggermode=FreeRun  triggersignal=1  trigsignalfromport=off  triggerlevel=0.0  triggerslope=Either  triggerscope=1  triggersample=0  filename=data.dat  mode=Lazy  writesize=512  autorestart=off  dynamicfilemode=off  maxwritefilesize=512*1024^2
  Scope 68 : slrtlib/Displays and Logging/Scope   scopeno=203  scopetype=Host  autostart=on  viewmode=Graphical redraw  formatstr='%15.6f'  grid=on  ylimits=[0,0]  nosamples=2500  noprepostsamples=0  interleave=1  triggermode=FreeRun  triggersignal=1  trigsignalfromport=off  triggerlevel=0.0  triggerslope=Either  triggerscope=1  triggersample=0  filename=data.dat  mode=Lazy  writesize=512  autorestart=off  dynamicfilemode=off  maxwritefilesize=512*1024^2
  Scope 69 : slrtlib/Displays and Logging/Scope   scopeno=204  scopetype=Host  autostart=on  viewmode=Graphical redraw  formatstr='%15.6f'  grid=on  ylimits=[0,0]  nosamples=2500  noprepostsamples=0  interleave=1  triggermode=FreeRun  triggersignal=1  trigsignalfromport=off  triggerlevel=0.0  triggerslope=Either  triggerscope=1  triggersample=0  filename=data.dat  mode=Lazy  writesize=512  autorestart=off  dynamicfilemode=off  maxwritefilesize=512*1024^2
  Scope 7 : slrtlib/Displays and Logging/Scope   scopeno=108  scopetype=Host  autostart=on  viewmode=Graphical redraw  formatstr='%15.6f'  grid=on  ylimits=[0,0]  nosamples=2500  noprepostsamples=0  interleave=1  triggermode=FreeRun  triggersignal=1  trigsignalfromport=off  triggerlevel=0.0  triggerslope=Either  triggerscope=1  triggersample=0  filename=data.dat  mode=Lazy  writesize=512  autorestart=off  dynamicfilemode=off  maxwritefilesize=512*1024^2
  Scope 70 : slrtlib/Displays and Logging/Scope   scopeno=205  scopetype=Host  autostart=on  viewmode=Graphical redraw  formatstr='%15.6f'  grid=on  ylimits=[0,0]  nosamples=2500  noprepostsamples=0  interleave=1  triggermode=FreeRun  triggersignal=1  trigsignalfromport=off  triggerlevel=0.0  triggerslope=Either  triggerscope=1  triggersample=0  filename=data.dat  mode=Lazy  writesize=512  autorestart=off  dynamicfilemode=off  maxwritefilesize=512*1024^2
  Scope 71 : slrtlib/Displays and Logging/Scope   scopeno=206  scopetype=Host  autostart=on  viewmode=Graphical redraw  formatstr='%15.6f'  grid=on  ylimits=[0,0]  nosamples=2500  noprepostsamples=0  interleave=1  triggermode=FreeRun  triggersignal=1  trigsignalfromport=off  triggerlevel=0.0  triggerslope=Either  triggerscope=1  triggersample=0  filename=data.dat  mode=Lazy  writesize=512  autorestart=off  dynamicfilemode=off  maxwritefilesize=512*1024^2
  Scope 72 : slrtlib/Displays and Logging/Scope   scopeno=207  scopetype=Host  autostart=on  viewmode=Graphical redraw  formatstr='%15.6f'  grid=on  ylimits=[0,0]  nosamples=2500  noprepostsamples=0  interleave=1  triggermode=FreeRun  triggersignal=1  trigsignalfromport=off  triggerlevel=0.0  triggerslope=Either  triggerscope=1  triggersample=0  filename=data.dat  mode=Lazy  writesize=512  autorestart=off  dynamicfilemode=off  maxwritefilesize=512*1024^2
  Scope 73 : slrtlib/Displays and Logging/Scope   scopeno=301  scopetype=Host  autostart=on  viewmode=Graphical redraw  formatstr='%15.6f'  grid=on  ylimits=[0,0]  nosamples=2500  noprepostsamples=0  interleave=1  triggermode=FreeRun  triggersignal=1  trigsignalfromport=off  triggerlevel=0.0  triggerslope=Either  triggerscope=1  triggersample=0  filename=data.dat  mode=Lazy  writesize=512  autorestart=off  dynamicfilemode=off  maxwritefilesize=512*1024^2
  Scope 74 : slrtlib/Displays and Logging/Scope   scopeno=302  scopetype=Host  autostart=on  viewmode=Graphical redraw  formatstr='%15.6f'  grid=on  ylimits=[0,0]  nosamples=2500  noprepostsamples=0  interleave=1  triggermode=FreeRun  triggersignal=1  trigsignalfromport=off  triggerlevel=0.0  triggerslope=Either  triggerscope=1  triggersample=0  filename=data.dat  mode=Lazy  writesize=512  autorestart=off  dynamicfilemode=off  maxwritefilesize=512*1024^2
  Scope 75 : slrtlib/Displays and Logging/Scope   scopeno=303  scopetype=Host  autostart=on  viewmode=Graphical redraw  formatstr='%15.6f'  grid=on  ylimits=[0,0]  nosamples=2500  noprepostsamples=0  interleave=1  triggermode=FreeRun  triggersignal=1  trigsignalfromport=off  triggerlevel=0.0  triggerslope=Either  triggerscope=1  triggersample=0  filename=data.dat  mode=Lazy  writesize=512  autorestart=off  dynamicfilemode=off  maxwritefilesize=512*1024^2
  Scope 76 : slrtlib/Displays and Logging/Scope   scopeno=304  scopetype=Host  autostart=on  viewmode=Graphical redraw  formatstr='%15.6f'  grid=on  ylimits=[0,0]  nosamples=2500  noprepostsamples=0  interleave=1  triggermode=FreeRun  triggersignal=1  trigsignalfromport=off  triggerlevel=0.0  triggerslope=Either  triggerscope=1  triggersample=0  filename=data.dat  mode=Lazy  writesize=512  autorestart=off  dynamicfilemode=off  maxwritefilesize=512*1024^2
  Scope 77 : slrtlib/Displays and Logging/Scope   scopeno=305  scopetype=Host  autostart=on  viewmode=Graphical redraw  formatstr='%15.6f'  grid=on  ylimits=[0,0]  nosamples=2500  noprepostsamples=0  interleave=1  triggermode=FreeRun  triggersignal=1  trigsignalfromport=off  triggerlevel=0.0  triggerslope=Either  triggerscope=1  triggersample=0  filename=data.dat  mode=Lazy  writesize=512  autorestart=off  dynamicfilemode=off  maxwritefilesize=512*1024^2
  Scope 78 : slrtlib/Displays and Logging/Scope   scopeno=306  scopetype=Host  autostart=on  viewmode=Graphical redraw  formatstr='%15.6f'  grid=on  ylimits=[0,0]  nosamples=2500  noprepostsamples=0  interleave=1  triggermode=FreeRun  triggersignal=1  trigsignalfromport=off  triggerlevel=0.0  triggerslope=Either  triggerscope=1  triggersample=0  filename=data.dat  mode=Lazy  writesize=512  autorestart=off  dynamicfilemode=off  maxwritefilesize=512*1024^2
  Scope 79 : slrtlib/Displays and Logging/Scope   scopeno=311  scopetype=Host  autostart=on  viewmode=Graphical redraw  formatstr='%15.6f'  grid=on  ylimits=[0,0]  nosamples=2500  noprepostsamples=0  interleave=1  triggermode=FreeRun  triggersignal=1  trigsignalfromport=off  triggerlevel=0.0  triggerslope=Either  triggerscope=1  triggersample=0  filename=data.dat  mode=Lazy  writesize=512  autorestart=off  dynamicfilemode=off  maxwritefilesize=512*1024^2
  Scope 8 : slrtlib/Displays and Logging/Scope   scopeno=109  scopetype=Host  autostart=on  viewmode=Graphical redraw  formatstr='%15.6f'  grid=on  ylimits=[0,0]  nosamples=2500  noprepostsamples=0  interleave=1  triggermode=FreeRun  triggersignal=1  trigsignalfromport=off  triggerlevel=0.0  triggerslope=Either  triggerscope=1  triggersample=0  filename=data.dat  mode=Lazy  writesize=512  autorestart=off  dynamicfilemode=off  maxwritefilesize=512*1024^2
  Scope 80 : slrtlib/Displays and Logging/Scope   scopeno=312  scopetype=Host  autostart=on  viewmode=Graphical redraw  formatstr='%15.6f'  grid=on  ylimits=[0,0]  nosamples=2500  noprepostsamples=0  interleave=1  triggermode=FreeRun  triggersignal=1  trigsignalfromport=off  triggerlevel=0.0  triggerslope=Either  triggerscope=1  triggersample=0  filename=data.dat  mode=Lazy  writesize=512  autorestart=off  dynamicfilemode=off  maxwritefilesize=512*1024^2
  Scope 81 : slrtlib/Displays and Logging/Scope   scopeno=313  scopetype=Host  autostart=on  viewmode=Graphical redraw  formatstr='%15.6f'  grid=on  ylimits=[0,0]  nosamples=2500  noprepostsamples=0  interleave=1  triggermode=FreeRun  triggersignal=1  trigsignalfromport=off  triggerlevel=0.0  triggerslope=Either  triggerscope=1  triggersample=0  filename=data.dat  mode=Lazy  writesize=512  autorestart=off  dynamicfilemode=off  maxwritefilesize=512*1024^2
  Scope 82 : slrtlib/Displays and Logging/Scope   scopeno=314  scopetype=Host  autostart=on  viewmode=Graphical redraw  formatstr='%15.6f'  grid=on  ylimits=[0,0]  nosamples=2500  noprepostsamples=0  interleave=1  triggermode=FreeRun  triggersignal=1  trigsignalfromport=off  triggerlevel=0.0  triggerslope=Either  triggerscope=1  triggersample=0  filename=data.dat  mode=Lazy  writesize=512  autorestart=off  dynamicfilemode=off  maxwritefilesize=512*1024^2
  Scope 83 : slrtlib/Displays and Logging/Scope   scopeno=315  scopetype=Host  autostart=on  viewmode=Graphical redraw  formatstr='%15.6f'  grid=on  ylimits=[0,0]  nosamples=2500  noprepostsamples=0  interleave=1  triggermode=FreeRun  triggersignal=1  trigsignalfromport=off  triggerlevel=0.0  triggerslope=Either  triggerscope=1  triggersample=0  filename=data.dat  mode=Lazy  writesize=512  autorestart=off  dynamicfilemode=off  maxwritefilesize=512*1024^2
  Scope 84 : slrtlib/Displays and Logging/Scope   scopeno=316  scopetype=Host  autostart=on  viewmode=Graphical redraw  formatstr='%15.6f'  grid=on  ylimits=[0,0]  nosamples=2500  noprepostsamples=0  interleave=1  triggermode=FreeRun  triggersignal=1  trigsignalfromport=off  triggerlevel=0.0  triggerslope=Either  triggerscope=1  triggersample=0  filename=data.dat  mode=Lazy  writesize=512  autorestart=off  dynamicfilemode=off  maxwritefilesize=512*1024^2
  Scope 85 : slrtlib/Displays and Logging/Scope   scopeno=211  scopetype=Host  autostart=on  viewmode=Graphical redraw  formatstr='%15.6f'  grid=on  ylimits=[0,0]  nosamples=2500  noprepostsamples=0  interleave=1  triggermode=FreeRun  triggersignal=1  trigsignalfromport=off  triggerlevel=0.0  triggerslope=Either  triggerscope=1  triggersample=0  filename=data.dat  mode=Lazy  writesize=512  autorestart=off  dynamicfilemode=off  maxwritefilesize=512*1024^2
  Scope 86 : slrtlib/Displays and Logging/Scope   scopeno=212  scopetype=Host  autostart=on  viewmode=Graphical redraw  formatstr='%15.6f'  grid=on  ylimits=[0,0]  nosamples=2500  noprepostsamples=0  interleave=1  triggermode=FreeRun  triggersignal=1  trigsignalfromport=off  triggerlevel=0.0  triggerslope=Either  triggerscope=1  triggersample=0  filename=data.dat  mode=Lazy  writesize=512  autorestart=off  dynamicfilemode=off  maxwritefilesize=512*1024^2
  Scope 87 : slrtlib/Displays and Logging/Scope   scopeno=213  scopetype=Host  autostart=on  viewmode=Graphical redraw  formatstr='%15.6f'  grid=on  ylimits=[0,0]  nosamples=2500  noprepostsamples=0  interleave=1  triggermode=FreeRun  triggersignal=1  trigsignalfromport=off  triggerlevel=0.0  triggerslope=Either  triggerscope=1  triggersample=0  filename=data.dat  mode=Lazy  writesize=512  autorestart=off  dynamicfilemode=off  maxwritefilesize=512*1024^2
  Scope 88 : slrtlib/Displays and Logging/Scope   scopeno=214  scopetype=Host  autostart=on  viewmode=Graphical redraw  formatstr='%15.6f'  grid=on  ylimits=[0,0]  nosamples=2500  noprepostsamples=0  interleave=1  triggermode=FreeRun  triggersignal=1  trigsignalfromport=off  triggerlevel=0.0  triggerslope=Either  triggerscope=1  triggersample=0  filename=data.dat  mode=Lazy  writesize=512  autorestart=off  dynamicfilemode=off  maxwritefilesize=512*1024^2
  Scope 89 : slrtlib/Displays and Logging/Scope   scopeno=215  scopetype=Host  autostart=on  viewmode=Graphical redraw  formatstr='%15.6f'  grid=on  ylimits=[0,0]  nosamples=2500  noprepostsamples=0  interleave=1  triggermode=FreeRun  triggersignal=1  trigsignalfromport=off  triggerlevel=0.0  triggerslope=Either  triggerscope=1  triggersample=0  filename=data.dat  mode=Lazy  writesize=512  autorestart=off  dynamicfilemode=off  maxwritefilesize=512*1024^2
  Scope 9 : slrtlib/Displays and Logging/Scope   scopeno=110  scopetype=Host  autostart=on  viewmode=Graphical redraw  formatstr='%15.6f'  grid=on  ylimits=[0,0]  nosamples=2500  noprepostsamples=0  interleave=1  triggermode=FreeRun  triggersignal=1  trigsignalfromport=off  triggerlevel=0.0  triggerslope=Either  triggerscope=1  triggersample=0  filename=data.dat  mode=Lazy  writesize=512  autorestart=off  dynamicfilemode=off  maxwritefilesize=512*1024^2
  Scope 90 : slrtlib/Displays and Logging/Scope   scopeno=216  scopetype=Host  autostart=on  viewmode=Graphical redraw  formatstr='%15.6f'  grid=on  ylimits=[0,0]  nosamples=2500  noprepostsamples=0  interleave=1  triggermode=FreeRun  triggersignal=1  trigsignalfromport=off  triggerlevel=0.0  triggerslope=Either  triggerscope=1  triggersample=0  filename=data.dat  mode=Lazy  writesize=512  autorestart=off  dynamicfilemode=off  maxwritefilesize=512*1024^2
  Scope 91 : slrtlib/Displays and Logging/Scope   scopeno=217  scopetype=Host  autostart=on  viewmode=Graphical redraw  formatstr='%15.6f'  grid=on  ylimits=[0,0]  nosamples=2500  noprepostsamples=0  interleave=1  triggermode=FreeRun  triggersignal=1  trigsignalfromport=off  triggerlevel=0.0  triggerslope=Either  triggerscope=1  triggersample=0  filename=data.dat  mode=Lazy  writesize=512  autorestart=off  dynamicfilemode=off  maxwritefilesize=512*1024^2
  Scope 92 : slrtlib/Displays and Logging/Scope   scopeno=218  scopetype=Host  autostart=on  viewmode=Graphical redraw  formatstr='%15.6f'  grid=on  ylimits=[0,0]  nosamples=2500  noprepostsamples=0  interleave=1  triggermode=FreeRun  triggersignal=1  trigsignalfromport=off  triggerlevel=0.0  triggerslope=Either  triggerscope=1  triggersample=0  filename=data.dat  mode=Lazy  writesize=512  autorestart=off  dynamicfilemode=off  maxwritefilesize=512*1024^2
  Scope 93 : slrtlib/Displays and Logging/Scope   scopeno=219  scopetype=Host  autostart=on  viewmode=Graphical redraw  formatstr='%15.6f'  grid=on  ylimits=[0,0]  nosamples=2500  noprepostsamples=0  interleave=1  triggermode=FreeRun  triggersignal=1  trigsignalfromport=off  triggerlevel=0.0  triggerslope=Either  triggerscope=1  triggersample=0  filename=data.dat  mode=Lazy  writesize=512  autorestart=off  dynamicfilemode=off  maxwritefilesize=512*1024^2
  Scope 94 : slrtlib/Displays and Logging/Scope   scopeno=220  scopetype=Host  autostart=on  viewmode=Graphical redraw  formatstr='%15.6f'  grid=on  ylimits=[0,0]  nosamples=2500  noprepostsamples=0  interleave=1  triggermode=FreeRun  triggersignal=1  trigsignalfromport=off  triggerlevel=0.0  triggerslope=Either  triggerscope=1  triggersample=0  filename=data.dat  mode=Lazy  writesize=512  autorestart=off  dynamicfilemode=off  maxwritefilesize=512*1024^2
  Scope 95 : slrtlib/Displays and Logging/Scope   scopeno=221  scopetype=Host  autostart=on  viewmode=Graphical redraw  formatstr='%15.6f'  grid=on  ylimits=[0,0]  nosamples=2500  noprepostsamples=0  interleave=1  triggermode=FreeRun  triggersignal=1  trigsignalfromport=off  triggerlevel=0.0  triggerslope=Either  triggerscope=1  triggersample=0  filename=data.dat  mode=Lazy  writesize=512  autorestart=off  dynamicfilemode=off  maxwritefilesize=512*1024^2
  Scope 96 : slrtlib/Displays and Logging/Scope   scopeno=222  scopetype=Host  autostart=on  viewmode=Graphical redraw  formatstr='%15.6f'  grid=on  ylimits=[0,0]  nosamples=2500  noprepostsamples=0  interleave=1  triggermode=FreeRun  triggersignal=1  trigsignalfromport=off  triggerlevel=0.0  triggerslope=Either  triggerscope=1  triggersample=0  filename=data.dat  mode=Lazy  writesize=512  autorestart=off  dynamicfilemode=off  maxwritefilesize=512*1024^2
  Scope 97 : slrtlib/Displays and Logging/Scope   scopeno=223  scopetype=Host  autostart=on  viewmode=Graphical redraw  formatstr='%15.6f'  grid=on  ylimits=[0,0]  nosamples=2500  noprepostsamples=0  interleave=1  triggermode=FreeRun  triggersignal=1  trigsignalfromport=off  triggerlevel=0.0  triggerslope=Either  triggerscope=1  triggersample=0  filename=data.dat  mode=Lazy  writesize=512  autorestart=off  dynamicfilemode=off  maxwritefilesize=512*1024^2
  Scope 98 : slrtlib/Displays and Logging/Scope   scopeno=224  scopetype=Host  autostart=on  viewmode=Graphical redraw  formatstr='%15.6f'  grid=on  ylimits=[0,0]  nosamples=2500  noprepostsamples=0  interleave=1  triggermode=FreeRun  triggersignal=1  trigsignalfromport=off  triggerlevel=0.0  triggerslope=Either  triggerscope=1  triggersample=0  filename=data.dat  mode=Lazy  writesize=512  autorestart=off  dynamicfilemode=off  maxwritefilesize=512*1024^2
  Scope 99 : slrtlib/Displays and Logging/Scope   scopeno=401  scopetype=Host  autostart=on  viewmode=Graphical redraw  formatstr='%15.6f'  grid=on  ylimits=[0,0]  nosamples=2500  noprepostsamples=0  interleave=1  triggermode=FreeRun  triggersignal=1  trigsignalfromport=off  triggerlevel=0.0  triggerslope=Either  triggerscope=1  triggersample=0  filename=data.dat  mode=Lazy  writesize=512  autorestart=off  dynamicfilemode=off  maxwritefilesize=512*1024^2
  Selector : Selector  InputPortWidth=10  IndexOptions=Index vector (dialog)  Indices=1  OutputSizes=1
  Selector1 : Selector  InputPortWidth=10  IndexOptions=Index vector (dialog)  Indices=1  OutputSizes=1
  Selector10 : Selector  InputPortWidth=10  IndexOptions=Index vector (dialog)  Indices=6  OutputSizes=1
  Selector100 : Selector  InputPortWidth=20  IndexOptions=Index vector (dialog)  Indices=6  OutputSizes=1
  Selector101 : Selector  InputPortWidth=20  IndexOptions=Index vector (dialog)  Indices=[12 19]  OutputSizes=1
  Selector102 : Selector  InputPortWidth=20  IndexOptions=Index vector (dialog)  Indices=[7 14]  OutputSizes=1
  Selector103 : Selector  InputPortWidth=20  IndexOptions=Index vector (dialog)  Indices=[8 15]  OutputSizes=1
  Selector104 : Selector  InputPortWidth=20  IndexOptions=Index vector (dialog)  Indices=[9 16]  OutputSizes=1
  Selector105 : Selector  InputPortWidth=20  IndexOptions=Index vector (dialog)  Indices=[10 17]  OutputSizes=1
  Selector106 : Selector  InputPortWidth=20  IndexOptions=Index vector (dialog)  Indices=[11 18]  OutputSizes=1
  Selector107 : Selector  InputPortWidth=20  IndexOptions=Index vector (dialog)  Indices=[13 20]  OutputSizes=1
  Selector108 : Selector  InputPortWidth=20  IndexOptions=Index vector (dialog)  Indices=[12 19]  OutputSizes=1
  Selector109 : Selector  InputPortWidth=20  IndexOptions=Index vector (dialog)  Indices=[7 14]  OutputSizes=1
  Selector11 : Selector  InputPortWidth=10  IndexOptions=Index vector (dialog)  Indices=6  OutputSizes=1
  Selector110 : Selector  InputPortWidth=20  IndexOptions=Index vector (dialog)  Indices=[8 15]  OutputSizes=1
  Selector111 : Selector  InputPortWidth=20  IndexOptions=Index vector (dialog)  Indices=[9 16]  OutputSizes=1
  Selector112 : Selector  InputPortWidth=20  IndexOptions=Index vector (dialog)  Indices=[10 17]  OutputSizes=1
  Selector113 : Selector  InputPortWidth=20  IndexOptions=Index vector (dialog)  Indices=[11 18]  OutputSizes=1
  Selector114 : Selector  InputPortWidth=20  IndexOptions=Index vector (dialog)  Indices=[13 20]  OutputSizes=1
  Selector115 : Selector  InputPortWidth=20  IndexOptions=Index vector (dialog)  Indices=12  OutputSizes=1
  Selector116 : Selector  InputPortWidth=20  IndexOptions=Index vector (dialog)  Indices=[7]  OutputSizes=1
  Selector117 : Selector  InputPortWidth=20  IndexOptions=Index vector (dialog)  Indices=8  OutputSizes=1
  Selector118 : Selector  InputPortWidth=20  IndexOptions=Index vector (dialog)  Indices=9  OutputSizes=1
  Selector119 : Selector  InputPortWidth=20  IndexOptions=Index vector (dialog)  Indices=10  OutputSizes=1
  Selector12 : Selector  InputPortWidth=10  IndexOptions=Index vector (dialog)  Indices=7  OutputSizes=1
  Selector120 : Selector  InputPortWidth=20  IndexOptions=Index vector (dialog)  Indices=11  OutputSizes=1
  Selector121 : Selector  InputPortWidth=20  IndexOptions=Index vector (dialog)  Indices=13  OutputSizes=1
  Selector122 : Selector  InputPortWidth=20  IndexOptions=Index vector (dialog)  Indices=19  OutputSizes=1
  Selector123 : Selector  InputPortWidth=20  IndexOptions=Index vector (dialog)  Indices=14  OutputSizes=1
  Selector124 : Selector  InputPortWidth=20  IndexOptions=Index vector (dialog)  Indices=15  OutputSizes=1
  Selector125 : Selector  InputPortWidth=20  IndexOptions=Index vector (dialog)  Indices=16  OutputSizes=1
  Selector126 : Selector  InputPortWidth=20  IndexOptions=Index vector (dialog)  Indices=17  OutputSizes=1
  Selector127 : Selector  InputPortWidth=20  IndexOptions=Index vector (dialog)  Indices=18  OutputSizes=1
  Selector128 : Selector  InputPortWidth=20  IndexOptions=Index vector (dialog)  Indices=20  OutputSizes=1
  Selector129 : Selector  InputPortWidth=20  IndexOptions=Index vector (dialog)  Indices=12  OutputSizes=1
  Selector13 : Selector  InputPortWidth=10  IndexOptions=Index vector (dialog)  Indices=7  OutputSizes=1
  Selector130 : Selector  InputPortWidth=20  IndexOptions=Index vector (dialog)  Indices=[7]  OutputSizes=1
  Selector131 : Selector  InputPortWidth=20  IndexOptions=Index vector (dialog)  Indices=8  OutputSizes=1
  Selector132 : Selector  InputPortWidth=20  IndexOptions=Index vector (dialog)  Indices=9  OutputSizes=1
  Selector133 : Selector  InputPortWidth=20  IndexOptions=Index vector (dialog)  Indices=10  OutputSizes=1
  Selector134 : Selector  InputPortWidth=20  IndexOptions=Index vector (dialog)  Indices=11  OutputSizes=1
  Selector135 : Selector  InputPortWidth=20  IndexOptions=Index vector (dialog)  Indices=13  OutputSizes=1
  Selector136 : Selector  InputPortWidth=20  IndexOptions=Index vector (dialog)  Indices=19  OutputSizes=1
  Selector137 : Selector  InputPortWidth=20  IndexOptions=Index vector (dialog)  Indices=14  OutputSizes=1
  Selector138 : Selector  InputPortWidth=20  IndexOptions=Index vector (dialog)  Indices=15  OutputSizes=1
  Selector139 : Selector  InputPortWidth=20  IndexOptions=Index vector (dialog)  Indices=16  OutputSizes=1
  Selector14 : Selector  InputPortWidth=10  IndexOptions=Index vector (dialog)  Indices=8  OutputSizes=1
  Selector140 : Selector  InputPortWidth=20  IndexOptions=Index vector (dialog)  Indices=17  OutputSizes=1
  Selector141 : Selector  InputPortWidth=20  IndexOptions=Index vector (dialog)  Indices=18  OutputSizes=1
  Selector142 : Selector  InputPortWidth=20  IndexOptions=Index vector (dialog)  Indices=20  OutputSizes=1
  Selector15 : Selector  InputPortWidth=10  IndexOptions=Index vector (dialog)  Indices=8  OutputSizes=1
  Selector16 : Selector  InputPortWidth=10  IndexOptions=Index vector (dialog)  Indices=9  OutputSizes=1
  Selector17 : Selector  InputPortWidth=10  IndexOptions=Index vector (dialog)  Indices=9  OutputSizes=1
  Selector18 : Selector  InputPortWidth=10  IndexOptions=Index vector (dialog)  Indices=10  OutputSizes=1
  Selector19 : Selector  InputPortWidth=10  IndexOptions=Index vector (dialog)  Indices=10  OutputSizes=1
  Selector2 : Selector  InputPortWidth=10  IndexOptions=Index vector (dialog)  Indices=2  OutputSizes=1
  Selector{20..21,28..29,52..53,68..69} (8 alike) : Selector  InputPortWidth=8  IndexOptions=Index vector (dialog)  Indices=1  OutputSizes=1
  Selector{22..23,30..31,54..55,70..71} (8 alike) : Selector  InputPortWidth=8  IndexOptions=Index vector (dialog)  Indices=6  OutputSizes=1
  Selector{24..25,40..41,56..57,73..74} (8 alike) : Selector  InputPortWidth=8  IndexOptions=Index vector (dialog)  Indices=7  OutputSizes=1
  Selector{26..27,42..43,58..59,75..76} (8 alike) : Selector  InputPortWidth=8  IndexOptions=Index vector (dialog)  Indices=8  OutputSizes=1
  Selector3 : Selector  InputPortWidth=10  IndexOptions=Index vector (dialog)  Indices=2  OutputSizes=1
  Selector{32..33,44..45,60..61,77..78} (8 alike) : Selector  InputPortWidth=8  IndexOptions=Index vector (dialog)  Indices=2  OutputSizes=1
  Selector{34..35,46..47,62..63,79..80} (8 alike) : Selector  InputPortWidth=8  IndexOptions=Index vector (dialog)  Indices=3  OutputSizes=1
  Selector{36..37,48..49,64..65,81..82} (8 alike) : Selector  InputPortWidth=8  IndexOptions=Index vector (dialog)  Indices=4  OutputSizes=1
  Selector{38..39,50..51,66..67,83..84} (8 alike) : Selector  InputPortWidth=8  IndexOptions=Index vector (dialog)  Indices=5  OutputSizes=1
  Selector4 : Selector  InputPortWidth=10  IndexOptions=Index vector (dialog)  Indices=3  OutputSizes=1
  Selector5 : Selector  InputPortWidth=10  IndexOptions=Index vector (dialog)  Indices=3  OutputSizes=1
  Selector6 : Selector  InputPortWidth=10  IndexOptions=Index vector (dialog)  Indices=4  OutputSizes=1
  Selector7 : Selector  InputPortWidth=10  IndexOptions=Index vector (dialog)  Indices=4  OutputSizes=1
  Selector72 : Selector  InputPortWidth=10  IndexOptions=Index vector (dialog)  Indices=[1,6]  OutputSizes=1
  Selector8 : Selector  InputPortWidth=10  IndexOptions=Index vector (dialog)  Indices=5  OutputSizes=1
  Selector85 : Selector  InputPortWidth=20  IndexOptions=Index vector (dialog)  Indices=1  OutputSizes=1
  Selector86 : Selector  InputPortWidth=20  IndexOptions=Index vector (dialog)  Indices=2  OutputSizes=1
  Selector87 : Selector  InputPortWidth=20  IndexOptions=Index vector (dialog)  Indices=3  OutputSizes=1
  Selector88 : Selector  InputPortWidth=20  IndexOptions=Index vector (dialog)  Indices=1  OutputSizes=1
  Selector89 : Selector  InputPortWidth=20  IndexOptions=Index vector (dialog)  Indices=2  OutputSizes=1
  Selector9 : Selector  InputPortWidth=10  IndexOptions=Index vector (dialog)  Indices=5  OutputSizes=1
  Selector90 : Selector  InputPortWidth=20  IndexOptions=Index vector (dialog)  Indices=3  OutputSizes=1
  Selector91 : Selector  InputPortWidth=20  IndexOptions=Index vector (dialog)  Indices=4  OutputSizes=1
  Selector92 : Selector  InputPortWidth=10  IndexOptions=Index vector (dialog)  Indices=[2 7]  OutputSizes=1
  Selector93 : Selector  InputPortWidth=20  IndexOptions=Index vector (dialog)  Indices=5  OutputSizes=1
  Selector94 : Selector  InputPortWidth=10  IndexOptions=Index vector (dialog)  Indices=[3 8]  OutputSizes=1
  Selector95 : Selector  InputPortWidth=20  IndexOptions=Index vector (dialog)  Indices=6  OutputSizes=1
  Selector96 : Selector  InputPortWidth=10  IndexOptions=Index vector (dialog)  Indices=[4 9]  OutputSizes=1
  Selector97 : Selector  InputPortWidth=20  IndexOptions=Index vector (dialog)  Indices=4  OutputSizes=1
  Selector98 : Selector  InputPortWidth=10  IndexOptions=Index vector (dialog)  Indices=[5 10]  OutputSizes=1
  Selector99 : Selector  InputPortWidth=20  IndexOptions=Index vector (dialog)  Indices=5  OutputSizes=1
  wires:
  Bus Selector/1 -> Gain10/1  "<qm0>"
  Bus Selector/2 -> Gain11/1  "<qmd>"
  Selector/1 -> Mux/1
  Selector1/1 -> Mux/2
  Mux/1 -> Reshape/1
  Selector3/1 -> Mux1/2
  Mux1/1 -> Reshape1/1
  Selector2/1 -> Mux1/1
  Selector5/1 -> Mux2/2
  Mux2/1 -> Reshape2/1
  Selector4/1 -> Mux2/1
  Selector7/1 -> Mux3/2
  Mux3/1 -> Reshape3/1
  Selector6/1 -> Mux3/1
  Selector9/1 -> Mux4/2
  Mux4/1 -> Reshape4/1
  Selector8/1 -> Mux4/1
  Mux8/1 -> Reshape8/1
  Selector15/1 -> Mux7/2
  Selector14/1 -> Mux7/1
  Selector18/1 -> Mux9/1
  Selector19/1 -> Mux9/2
  Selector13/1 -> Mux6/2
  Selector12/1 -> Mux6/1
  Selector17/1 -> Mux8/2
  Mux7/1 -> Reshape7/1
  Mux6/1 -> Reshape6/1
  Selector11/1 -> Mux5/2
  Mux5/1 -> Reshape5/1
  Mux9/1 -> Reshape9/1
  Selector16/1 -> Mux8/1
  Selector10/1 -> Mux5/1
  Reshape/1 -> "Scope "/1, Scope/1
  Reshape1/1 -> Scope 1/1, Scope1/1
  Reshape2/1 -> Scope 2/1, Scope2/1
  Reshape3/1 -> Scope 3/1, Scope3/1
  Reshape4/1 -> Scope 4/1, Scope4/1
  Reshape5/1 -> Scope 5/1, Scope5/1
  Reshape8/1 -> Scope 8/1, Scope8/1
  Reshape9/1 -> Scope9/1, Scope 9/1
  Reshape6/1 -> Scope 6/1, Scope6/1
  Reshape7/1 -> Scope 7/1, Scope7/1
  Mux13/1 -> Reshape13/1
  Selector35/1 -> Mux12/2
  Selector34/1 -> Mux12/1
  Reshape16/1 -> Scope 16/1, Scope16/1
  Selector39/1 -> Mux14/2
  Reshape11/1 -> Scope 11/1, Scope11/1
  Selector38/1 -> Mux14/1
  Reshape15/1 -> Scope 15/1, Scope15/1
  Reshape12/1 -> Scope 12/1, Scope12/1
  Bus Selector2/1 -> Selector38/1, Selector26/1, Selector24/1, Selector22/1, Selector36/1, Selector34/1, Selector32/1, Selector20/1  "<hr>"
  Mux16/1 -> Reshape16/1
  Mux17/1 -> Reshape17/1
  Mux15/1 -> Reshape15/1
  Selector33/1 -> Mux11/2
  Reshape14/1 -> Scope 14/1, Scope14/1
  Mux12/1 -> Reshape12/1
  Selector32/1 -> Mux11/1
  Selector22/1 -> Mux15/1
  Mux14/1 -> Reshape14/1
  Selector24/1 -> Mux16/1
  Selector25/1 -> Mux16/2
  Bus Selector2/2 -> Selector37/1, Selector39/1, Selector27/1, Selector25/1, Selector23/1, Selector35/1, Selector33/1, Selector21/1  "<h0>"
  Selector37/1 -> Mux13/2
  Selector23/1 -> Mux15/2
  Mux11/1 -> Reshape11/1
  Reshape13/1 -> Scope 13/1, Scope13/1
  Selector26/1 -> Mux17/1
  Selector21/1 -> Mux10/2
  Mux10/1 -> Reshape10/1
  Selector36/1 -> Mux13/1
  Selector20/1 -> Mux10/1
  Reshape10/1 -> Scope 10/1, Scope10/1
  Selector27/1 -> Mux17/2
  Reshape17/1 -> Scope 17/1, Scope17/1
  Selector43/1 -> Mux25/2
  Reshape25/1 -> Scope 25/1, Scope25/1
  Reshape18/1 -> Scope 18/1, Scope18/1
  Selector28/1 -> Mux18/1
  Mux18/1 -> Reshape18/1
  Selector42/1 -> Mux25/1
  Selector49/1 -> Mux21/2
  Selector31/1 -> Mux23/2
  Selector40/1 -> Mux24/1
  Selector29/1 -> Mux18/2
  Selector30/1 -> Mux23/1
  Selector41/1 -> Mux24/2
  Selector45/1 -> Mux19/2
  Mux20/1 -> Reshape20/1
  Mux23/1 -> Reshape23/1
  Mux25/1 -> Reshape25/1
  Mux24/1 -> Reshape24/1
  Reshape21/1 -> Scope 21/1, Scope21/1
  Selector51/1 -> Mux22/2
  Reshape20/1 -> Scope 20/1, Scope20/1
  Mux21/1 -> Reshape21/1
  Selector48/1 -> Mux21/1
  Selector46/1 -> Mux20/1
  Reshape23/1 -> Scope 23/1, Scope23/1
  Mux22/1 -> Reshape22/1
  Bus Selector3/2 -> Gain13/1  "<q0_control>"
  Selector50/1 -> Mux22/1
  Mux19/1 -> Reshape19/1
  Reshape24/1 -> Scope 24/1, Scope24/1
  Reshape19/1 -> Scope 19/1, Scope19/1
  Bus Selector3/1 -> Gain12/1  "<qd_control>"
  Selector44/1 -> Mux19/1
  Selector47/1 -> Mux20/2
  Reshape22/1 -> Scope 22/1, Scope22/1
  Bus Selector4/2 -> Gain15/1  "<dq0_control>"
  Selector60/1 -> Mux27/1
  Reshape30/1 -> Scope 30/1, Scope30/1
  Selector63/1 -> Mux28/2
  Mux27/1 -> Reshape27/1
  Selector66/1 -> Mux30/1
  Bus Selector4/1 -> Gain14/1  "<dqd_control>"
  Mux29/1 -> Reshape29/1
  Mux30/1 -> Reshape30/1
  Reshape28/1 -> Scope 28/1, Scope28/1
  Mux32/1 -> Reshape32/1
  Mux31/1 -> Reshape31/1
  Mux33/1 -> Reshape33/1
  Selector62/1 -> Mux28/1
  Reshape29/1 -> Scope 29/1, Scope29/1
  Reshape31/1 -> Scope 31/1, Scope31/1
  Selector64/1 -> Mux29/1
  Selector67/1 -> Mux30/2
  Selector65/1 -> Mux29/2
  Selector61/1 -> Mux27/2
  Selector55/1 -> Mux31/2
  Selector53/1 -> Mux26/2
  Selector57/1 -> Mux32/2
  Selector58/1 -> Mux33/1
  Reshape26/1 -> Scope 26/1, Scope26/1
  Selector59/1 -> Mux33/2
  Reshape32/1 -> Scope 32/1, Scope32/1
  Selector54/1 -> Mux31/1
  Reshape33/1 -> Scope 33/1, Scope33/1
  Selector52/1 -> Mux26/1
  Selector56/1 -> Mux32/1
  Reshape27/1 -> Scope 27/1, Scope27/1
  Mux26/1 -> Reshape26/1
  Mux28/1 -> Reshape28/1
  Bus Selector5/1 -> Selector92/1, Selector72/1, Selector98/1, Selector96/1, Selector94/1  "<u>"
  Selector96/1 -> Reshape43/1
  Reshape41/1 -> Scope 41/1, Scope41/1
  Reshape42/1 -> Scope 42/1, Scope42/1
  Reshape44/1 -> Scope34/1, Scope 44/1
  Selector94/1 -> Reshape42/1
  Selector98/1 -> Reshape44/1
  Selector92/1 -> Reshape41/1
  Reshape43/1 -> Scope 43/1, Scope43/1
  Selector72/1 -> Reshape40/1
  Reshape40/1 -> Scope 40/1, Scope40/1
  Bus Selector1/2 -> Selector69/1, Selector82/1, Selector84/1, Selector76/1, Selector74/1, Selector71/1, Selector80/1, Selector78/1  "<hr_recover>"
  Bus Selector1/1 -> Selector68/1, Selector83/1, Selector75/1, Selector73/1, Selector70/1, Selector81/1, Selector79/1, Selector77/1  "<hr>"
  Reshape35/1 -> Scope 35/1, Scope36/1
  Mux34/1 -> Reshape34/1
  Mux36/1 -> Reshape36/1
  Selector68/1 -> Mux34/1
  Selector70/1 -> Mux39/1
  Selector76/1 -> Mux41/2
  Reshape45/1 -> Scope 45/1, Scope45/1
  Selector69/1 -> Mux34/2
  Reshape34/1 -> Scope 34/1, Scope35/1
  Mux41/1 -> Reshape46/1
  Selector81/1 -> Mux37/1
  Reshape39/1 -> Scope 39/1, Scope44/1
  Selector73/1 -> Mux40/1
  Reshape37/1 -> Scope 37/1, Scope38/1
  Selector79/1 -> Mux36/1
  Selector84/1 -> Mux38/2
  Selector78/1 -> Mux35/2
  Selector75/1 -> Mux41/1
  Mux39/1 -> Reshape39/1
  Selector74/1 -> Mux40/2
  Mux40/1 -> Reshape45/1
  Selector71/1 -> Mux39/2
  Mux38/1 -> Reshape38/1
  Mux37/1 -> Reshape37/1
  Reshape46/1 -> Scope 46/1, Scope46/1
  Selector77/1 -> Mux35/1
  Reshape38/1 -> Scope 38/1, Scope39/1
  Selector80/1 -> Mux36/2
  Selector83/1 -> Mux38/1
  Reshape36/1 -> Scope 36/1, Scope37/1
  Mux35/1 -> Reshape35/1
  Selector82/1 -> Mux37/2
  Bus Selector6/1 -> Gain16/1  "<q>"
  Selector85/1 -> Reshape47/1
  Reshape47/1 -> Scope 47/1, Scope47/1
  Selector86/1 -> Reshape48/1
  Reshape48/1 -> Scope 48/1, Scope48/1
  Selector87/1 -> Reshape49/1
  Reshape49/1 -> Scope 49/1, Scope49/1
  Selector88/1 -> Reshape50/1
  Reshape51/1 -> Scope 51/1, Scope51/1
  Reshape50/1 -> Scope 50/1, Scope50/1
  Reshape52/1 -> Scope 52/1, Scope52/1
  Selector89/1 -> Reshape51/1
  Selector90/1 -> Reshape52/1
  Bus Selector6/2 -> Gain17/1  "<dq>"
  Bus Selector7/1 -> Gain18/1  "<q>"
  Selector91/1 -> Reshape53/1
  Reshape54/1 -> Scope 54/1, Scope54/1
  Selector93/1 -> Reshape54/1
  Reshape58/1 -> Scope 58/1, Scope58/1
  Reshape56/1 -> Scope 56/1, Scope56/1
  Selector100/1 -> Reshape58/1
  Selector99/1 -> Reshape57/1
  Bus Selector7/2 -> Gain19/1  "<dq>"
  Reshape57/1 -> Scope 57/1, Scope57/1
  Selector97/1 -> Reshape56/1
  Reshape53/1 -> Scope 53/1, Scope53/1
  Selector95/1 -> Reshape55/1
  Reshape55/1 -> Scope 55/1, Scope55/1
  Selector102/1 -> Reshape59/1
  Reshape59/1 -> Scope 59/1, Scope59/1
  Reshape60/1 -> Scope 60/1, Scope60/1
  Reshape61/1 -> Scope 61/1, Scope61/1
  Reshape63/1 -> Scope 63/1, Scope63/1
  Selector105/1 -> Reshape62/1
  Selector104/1 -> Reshape61/1
  Selector106/1 -> Reshape63/1
  Selector101/1 -> Reshape64/1
  Reshape62/1 -> Scope 62/1, Scope62/1
  Reshape64/1 -> Scope 64/1, Scope64/1
  Selector103/1 -> Reshape60/1
  Reshape65/1 -> Scope 65/1, Scope65/1
  Selector107/1 -> Reshape65/1
  Bus Selector8/1 -> Gain20/1  "<q>"
  Selector109/1 -> Reshape66/1
  Reshape69/1 -> Scope 69/1, Scope69/1
  Selector110/1 -> Reshape67/1
  Bus Selector8/2 -> Gain21/1  "<dq>"
  Selector111/1 -> Reshape68/1
  Selector108/1 -> Reshape71/1
  Selector113/1 -> Reshape70/1
  Reshape72/1 -> Scope 72/1, Scope72/1
  Selector112/1 -> Reshape69/1
  Selector114/1 -> Reshape72/1
  Reshape70/1 -> Scope 70/1, Scope70/1
  Reshape67/1 -> Scope 67/1, Scope67/1
  Reshape71/1 -> Scope 71/1, Scope71/1
  Reshape66/1 -> Scope 66/1, Scope66/1
  Reshape68/1 -> Scope 68/1, Scope68/1
  In1/1 -> Bus Selector10/1, Bus Selector9/1, Bus Selector11/1, Bus Selector/1, Bus Selector2/1, Bus Selector3/1, Bus Selector4/1, Bus Selector5/1, Bus Selector6/1, Bus Selector12/1, Bus Selector8/1, Bus Selector7/1, Bus Selector1/1
  Bus Selector9/4 -> Mux43/2, Reshape76/1  "<Ly_stToe_stTD0_kf>"
  Reshape73/1 -> Scope 73/1, Scope73/1
  Bus Selector9/3 -> Mux42/2, Reshape75/1  "<Lx_stToe_stTD0_kf>"
  Reshape76/1 -> Scope 76/1, Scope76/1
  Bus Selector9/2 -> Reshape74/1, Mux43/1  "<Ly_stToe_stTD0_obs>"
  Reshape75/1 -> Scope 75/1, Scope75/1
  Bus Selector9/1 -> Mux42/1, Reshape73/1  "<Lx_stToe_stTD0_obs>"
  Reshape74/1 -> Scope 74/1, Scope74/1
  Reshape77/1 -> Scope 77/1, Scope77/1
  Reshape78/1 -> Scope 78/1, Scope78/1
  Mux42/1 -> Reshape77/1
  Mux43/1 -> Reshape78/1
  Reshape80/1 -> Scope 80/1, Scope80/1
  Reshape82/1 -> Scope 82/1, Scope82/1
  Reshape81/1 -> Scope 81/1, Scope81/1
  Bus Selector10/3 -> Gain3/1  "<rp_LToe_fil>"
  Bus Selector10/4 -> Gain4/1  "<rp_RToe_fil>"
  Bus Selector10/1 -> Gain1/1  "<rp_LToe>"
  Reshape84/1 -> Scope 84/1, Scope84/1
  Reshape79/1 -> Scope 79/1, Scope79/1
  Mux44/1 -> Reshape83/1
  Mux45/1 -> Reshape84/1
  Bus Selector10/2 -> Gain2/1  "<rp_RToe>"
  Reshape83/1 -> Scope 83/1, Scope83/1
  Bus Selector12/1 -> Gain22/1  "<dq>"
  Bus Selector12/2 -> Gain23/1  "<dq_ss>"
  Selector116/1 -> Mux46/1
  Selector130/1 -> Mux46/2
  Selector131/1 -> Mux47/2
  Selector117/1 -> Mux47/1
  Selector132/1 -> Mux48/2
  Selector118/1 -> Mux48/1
  Selector133/1 -> Mux49/2
  Selector119/1 -> Mux49/1
  Selector134/1 -> Mux50/2
  Selector120/1 -> Mux50/1
  Selector129/1 -> Mux51/2
  Selector115/1 -> Mux51/1
  Selector135/1 -> Mux52/2
  Selector121/1 -> Mux52/1
  Mux46/1 -> Reshape85/1
  Reshape85/1 -> Scope 85/1, Scope85/1
  Reshape86/1 -> Scope 86/1, Scope86/1
  Mux47/1 -> Reshape86/1
  Reshape87/1 -> Scope 87/1, Scope87/1
  Mux48/1 -> Reshape87/1
  Reshape88/1 -> Scope 88/1, Scope88/1
  Mux49/1 -> Reshape88/1
  Reshape89/1 -> Scope 89/1, Scope89/1
  Mux50/1 -> Reshape89/1
  Reshape90/1 -> Scope 90/1, Scope90/1
  Mux51/1 -> Reshape90/1
  Reshape91/1 -> Scope 91/1, Scope91/1
  Mux52/1 -> Reshape91/1
  Reshape92/1 -> Scope 92/1, Scope92/1
  Mux53/1 -> Reshape92/1
  Selector123/1 -> Mux53/1
  Selector137/1 -> Mux53/2
  Reshape93/1 -> Scope 93/1, Scope93/1
  Mux54/1 -> Reshape93/1
  Selector124/1 -> Mux54/1
  Selector138/1 -> Mux54/2
  Reshape94/1 -> Scope 94/1, Scope94/1
  Mux55/1 -> Reshape94/1
  Selector125/1 -> Mux55/1
  Selector139/1 -> Mux55/2
  Selector142/1 -> Mux59/2
  Selector141/1 -> Mux57/2
  Mux57/1 -> Reshape96/1
  Reshape96/1 -> Scope 96/1, Scope96/1
  Mux56/1 -> Reshape95/1
  Mux58/1 -> Reshape97/1
  Reshape97/1 -> Scope 97/1, Scope97/1
  Reshape95/1 -> Scope 95/1, Scope95/1
  Selector136/1 -> Mux58/2
  Selector128/1 -> Mux59/1
  Selector126/1 -> Mux56/1
  Selector140/1 -> Mux56/2
  Mux59/1 -> Reshape98/1
  Selector127/1 -> Mux57/1
  Reshape98/1 -> Scope 98/1, Scope98/1
  Selector122/1 -> Mux58/1
  Bus Selector11/1 -> Gain9/1  "<s>"
  Reshape99/1 -> Scope 99/1, Scope99/1
  In2/1 -> Bus Selector14/1, Bus Selector13/1
  Demux/3 -> Reshape102/1
  Demux/2 -> Reshape101/1
  Reshape102/1 -> Scope 102/1, Scope102/1
  Demux/1 -> Reshape100/1
  Reshape100/1 -> Scope 100/1, Scope100/1
  Reshape101/1 -> Scope 101/1, Scope101/1
  Bus Selector11/2 -> Gain8/1  "<qsL_1>"
  Bus Selector11/3 -> Gain7/1  "<qsR_1>"
  Reshape103/1 -> Scope 103/1, Scope103/1
  Mux60/1 -> Reshape103/1
  Mux61/1 -> Reshape104/1
  Bus Selector11/5 -> Gain5/1  "<qsR_2>"
  Reshape104/1 -> Scope 104/1, Scope104/1
  Bus Selector11/4 -> Gain6/1  "<qsL_2>"
  Bus Selector13/1 -> Gain/1  "<a_world>"
  Gain/1 -> Demux/1
  Gain1/1 -> Mux44/1, Reshape79/1
  Gain2/1 -> Reshape80/1, Mux45/1
  Gain3/1 -> Mux44/2, Reshape81/1
  Gain4/1 -> Mux45/2, Reshape82/1
  Gain5/1 -> Mux61/2
  Gain6/1 -> Mux61/1
  Gain7/1 -> Mux60/2
  Gain8/1 -> Mux60/1
  Gain9/1 -> Reshape99/1
  Gain10/1 -> Selector8/1, Selector18/1, Selector16/1, Selector14/1, Selector12/1, Selector10/1, Selector6/1, Selector4/1, Selector2/1, Selector/1
  Gain11/1 -> Selector7/1, Selector9/1, Selector19/1, Selector17/1, Selector15/1, Selector13/1, Selector11/1, Selector5/1, Selector3/1, Selector1/1
  Gain12/1 -> Selector50/1, Selector42/1, Selector40/1, Selector30/1, Selector48/1, Selector46/1, Selector44/1, Selector28/1
  Gain13/1 -> Selector49/1, Selector51/1, Selector43/1, Selector41/1, Selector31/1, Selector47/1, Selector45/1, Selector29/1
  Gain14/1 -> Selector52/1, Selector66/1, Selector58/1, Selector56/1, Selector54/1, Selector64/1, Selector62/1, Selector60/1
  Gain15/1 -> Selector53/1, Selector65/1, Selector67/1, Selector59/1, Selector57/1, Selector55/1, Selector63/1, Selector61/1
  Gain16/1 -> Selector86/1, Selector87/1, Selector85/1
  Gain17/1 -> Selector90/1, Selector89/1, Selector88/1
  Gain18/1 -> Selector93/1, Selector95/1, Selector91/1
  Gain19/1 -> Selector100/1, Selector99/1, Selector97/1
  Gain20/1 -> Selector107/1, Selector101/1, Selector106/1, Selector105/1, Selector104/1, Selector103/1, Selector102/1
  Gain21/1 -> Selector114/1, Selector108/1, Selector113/1, Selector112/1, Selector111/1, Selector110/1, Selector109/1
  Gain22/1 -> Selector128/1, Selector122/1, Selector127/1, Selector126/1, Selector125/1, Selector124/1, Selector123/1, Selector121/1, Selector115/1, Selector120/1, Selector119/1, Selector118/1, Selector117/1, Selector116/1
  Gain23/1 -> Selector142/1, Selector136/1, Selector141/1, Selector140/1, Selector139/1, Selector138/1, Selector137/1, Selector135/1, Selector129/1, Selector134/1, Selector133/1, Selector132/1, Selector131/1, Selector130/1
  Bus Selector14/1 -> Gain24/1  "<ITx_kf>"
  Reshape107/1 -> Scope 107/1, Scope107/1
  Reshape106/1 -> Scope 106/1, Scope106/1
  Reshape105/1 -> Scope 105/1, Scope105/1
  Demux1/2 -> Reshape106/1
  Demux1/1 -> Reshape105/1
  Demux1/3 -> Reshape107/1
  Demux1/4 -> Reshape108/1
  Reshape108/1 -> Scope 108/1, Scope108/1
  Gain24/1 -> Demux1/1
  Demux2/4 -> Reshape112/1
  Demux2/1 -> Reshape109/1
  Demux2/3 -> Reshape111/1
  Demux2/2 -> Reshape110/1
  Reshape112/1 -> Scope 112/1, Scope112/1
  Reshape110/1 -> Scope 110/1, Scope110/1
  Reshape111/1 -> Scope 111/1, Scope111/1
  Gain25/1 -> Demux2/1
  Bus Selector14/2 -> Gain25/1  "<ITy_kf>"
  Reshape109/1 -> Scope 109/1, Scope109/1
  Demux3/4 -> Reshape116/1
  Demux3/1 -> Reshape113/1
  Demux3/3 -> Reshape115/1
  Demux3/2 -> Reshape114/1
  Reshape116/1 -> Scope 116/1, Scope116/1
  Reshape114/1 -> Scope 114/1, Scope114/1
  Reshape115/1 -> Scope 115/1, Scope115/1
  Gain26/1 -> Demux3/1
  Bus Selector14/3 -> Gain26/1  "<ITz_kf>"
  Reshape113/1 -> Scope 113/1, Scope113/1
